simulink library "pneAux_rebuild_generic_std"  (R2016a)
settings: Solver=VariableStepAuto  StartTime=0.0  StopTime=10.0  RelTol=1e-3
undefined symbols (not defined in the file): sMP
(part 1 of 2)
settings Model: Creator=CAB  LastModifiedBy=CAB
settings GRTTargetCC: GeneratePreprocessorConditionals=Use local settings

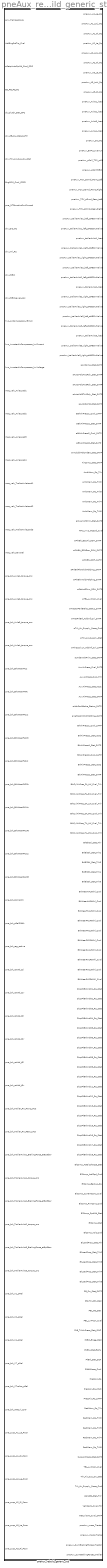
== system pneAux_rebuild_generic_std ==
  pneAux_rebuild_generic_std : Subsystem  mask{s1=sMP.ctrl.pneAux.settings_iMode, s2=sMP.ctrl.pneAux.settings_dt, initCmd='Parameters_pneAux_rebuild_generic_std_sf', p1=sMP.ctrl.pneAux.out.aAirComp_Stat_SATP, p2=sMP.ctrl.pneAux.out.aAutoMd1To2Rdy_Stat_SATP, p3=sMP.ctrl.pneAux.out.aAutoMd1To3Rdy_Stat_SATP, p4=sMP.ctrl.pneAux.out.aAutoMd3To1Rdy_Stat_SATP, p5=sMP.ctrl.pneAux.out.aAutoOpMd_Stat_SATP, p6=sMP.ctrl.pneAux.out.aBrkAirPress1_Cval_SATP, p7=sMP.ctrl.pneAux.out.aBrkAirPress1_Stat_SATP, p8=sMP.ctrl.pneAux.out.aBrkAirPress2_Cval_SATP, p9=sMP.ctrl.pneAux.out.aBrkAirPress2_Stat_SATP, p10=sMP.ctrl.pneAux.in.ActlEngPctTrq_Cval, p11=sMP.ctrl.pneAux.out.aImplsblMdCmdErr_Stat_SATP, p12=sMP.ctrl.pneAux.out.AirComp_Stat_SATP, p13=sMP.ctrl.pneAux.out.AmbWarn_Rq_Trlr2, p14=sMP.ctrl.pneAux.out.AmbWarn_Rq_Trlr3, p15=sMP.ctrl.pneAux.out.AmbWarn_Rq_Trlr4, p16=sMP.ctrl.pneAux.out.AmbWarn_Rq_Trlr5, p17=sMP.ctrl.pneAux.out.AmbWarn_Rq_Trlr, p18=sMP.ctrl.pneAux.out.aOverVoltPrim_Stat_SATP, p19=sMP.ctrl.pneAux.out.API2_Inv2_RqSpd_Cval, p20=sMP.ctrl.pneAux.out.aPrkBrk_ECUAir_SOH_SATP, p21=sMP.ctrl.pneAux.out.aPrkBrk_ECUGen_SOH_SATP, p22=sMP.ctrl.pneAux.out.aPrkBrk_SOH_SATP, p23=sMP.ctrl.pneAux.out.aPrkBrkFltIntrlckMdChng_SATP, p24=sMP.ctrl.pneAux.out.aPrkBrkIntrlckMdChng_SATP, p25=sMP.ctrl.pneAux.in.aSatpAutoOpMd_Cmd_SDS, p26=sMP.ctrl.pneAux.out.aSdsIntfPrim_SOH_SATP, p27=sMP.ctrl.pneAux.out.aTBL_LvrPosn_Cval, p28=sMP.ctrl.pneAux.ATBVehicleParameter, p29=sMP.ctrl.pneAux.out.aTractorParkBrake_Status_SATP, p30=sMP.ctrl.pneAux.out.aTrctrPrkBrk_AddInf_Cvl_SATP, p31=sMP.ctrl.pneAux.out.aTrlr_Air_Supply_Press_Cval, p32=sMP.ctrl.pneAux.out.aTrlr_Air_Supply_Stat, p33=sMP.ctrl.pneAux.out.aTrlrSpplyLn_AddInf_Cvl_SATP, p34=sMP.ctrl.pneAux.out.aUnderVoltPrim_Stat_SATP, p35=sMP.ctrl.pneAux.out.AuxAirPress_Cval_SATP, p36=sMP.ctrl.pneAux.out.AuxAirPress_Cval_Trlr, p37=sMP.ctrl.pneAux.out.AuxAirPress_Stat_ICUC, p38=sMP.ctrl.pneAux.out.AuxAirPress_Stat_SATP, p39=sMP.ctrl.pneAux.out.aVehParkBrake_Status_SATP, p40=sMP.ctrl.pneAux.out.aVehSpdIntrlckMdChng_SATP, p41=sMP.ctrl.pneAux.out.BrkAirPress1_Cval_SATP, p42=sMP.ctrl.pneAux.out.BrkAirPress1_Stat_ICUC, p43=sMP.ctrl.pneAux.out.BrkAirPress1_Stat_SATP, p44=sMP.ctrl.pneAux.out.BrkAirPress2_Cval_SATP, p45=sMP.ctrl.pneAux.out.BrkAirPress2_Stat_ICUC, p46=sMP.ctrl.pneAux.out.BrkAirPress2_Stat_SATP, p47=sMP.ctrl.pneAux.out.BrkCylAirPres_FA_LW_Cval_Trlr, p48=sMP.ctrl.pneAux.out.BrkCylAirPres_FA_RW_Cval_Trlr, p49=sMP.ctrl.pneAux.out.BrkCylAirPres_SA_LW_Cval_Trlr, p50=sMP.ctrl.pneAux.out.BrkCylAirPres_SA_RW_Cval_Trlr, p51=sMP.ctrl.pneAux.out.BrkCylAirPres_TA_LW_Cval_Trlr, p52=sMP.ctrl.pneAux.out.BrkCylAirPres_TA_RW_Cval_Trlr, p53=sMP.ctrl.pneAux.out.BrkElCtrl_Stat_Trlr2, p54=sMP.ctrl.pneAux.out.BrkElCtrl_Stat_Trlr3, p55=sMP.ctrl.pneAux.out.BrkElCtrl_Stat_Trlr4, p56=sMP.ctrl.pneAux.out.BrkElCtrl_Stat_Trlr5, p57=sMP.ctrl.pneAux.out.BrkElCtrl_Stat_Trlr, p58=sMP.ctrl.pneAux.out.BrkWearAALtWhl_Cval, p59=sMP.ctrl.pneAux.out.BrkWearAARtWhl_Cval, p60=sMP.ctrl.pneAux.out.BrkWearFA1LtWhl_Cval, p61=sMP.ctrl.pneAux.out.BrkWearFA1RtWhl_Cval, p62=sMP.ctrl.pneAux.out.BrkWearFA2LtWhl_Cval, p63=sMP.ctrl.pneAux.out.BrkWearFA2RtWhl_Cval, p64=sMP.ctrl.pneAux.out.BrkWearRA1LtWhl_Cval, p65=sMP.ctrl.pneAux.out.BrkWearRA1RtWhl_Cval, p66=sMP.ctrl.pneAux.out.BrkWearRA2LtWhl_Cval, p67=sMP.ctrl.pneAux.out.BrkWearRA2RtWhl_Cval, p68=sMP.ctrl.pneAux.in.BS_PB_Fct_Rq, p69=sMP.ctrl.pneAux.in.ch_Clutch_Stat_CPC, p70=sMP.ctrl.pneAux.out.DispPkBrkInd01_Rq_Stat, p71=sMP.ctrl.pneAux.out.DispPkBrkInd02_Rq_Stat, p72=sMP.ctrl.pneAux.out.DispPkBrkInd03_Rq_Stat, p73=sMP.ctrl.pneAux.out.DispPkBrkInd04_Rq_Stat, p74=sMP.ctrl.pneAux.out.DispPkBrkInd05_Rq_Stat, p75=sMP.ctrl.pneAux.out.DispPkBrkInd06_Rq_Stat, p76=sMP.ctrl.pneAux.out.DispPkBrkInd07_Rq_Stat, p77=sMP.ctrl.pneAux.out.DispPkBrkInd08_Rq_Stat, p78=sMP.ctrl.pneAux.out.DispPkBrkInd09_Rq_Stat, p79=sMP.ctrl.pneAux.out.DispPkBrkInd10_Rq_Stat, p80=sMP.ctrl.pneAux.out.DispPkBrkInd11_Rq_Stat, p81=sMP.ctrl.pneAux.out.DispPkBrkInd12_Rq_Stat, p82=sMP.ctrl.pneAux.out.DispPkBrkInd13_Rq_Stat, p83=sMP.ctrl.pneAux.out.DispPkBrkInd14_Rq_Stat, p84=sMP.ctrl.pneAux.out.DispPkBrkInd15_Rq_Stat, p85=sMP.ctrl.pneAux.out.DispPkBrkInd16_Rq_Stat, p86=sMP.ctrl.pneAux.out.DispPkBrkInd17_Rq_Stat, p87=sMP.ctrl.pneAux.out.DispPkBrkInd18_Rq_Stat, p88=sMP.ctrl.pneAux.in.drv_DrS_Rq, p89=sMP.ctrl.pneAux.in.drv_Knl_Rq, p90=sMP.ctrl.pneAux.in.drv_PB_Sw_Stat_SATP, p91=sMP.ctrl.pneAux.in.drv_PkBrk, p92=sMP.ctrl.pneAux.in.drv_PkBrkLever_pos, p93=sMP.ctrl.pneAux.in.drv_Trlr_Air_Sup_Sw_Stat, p94=sMP.ctrl.pneAux.out.ElComp_ActDischarge_Stat, p95=sMP.ctrl.pneAux.out.ElComp_ActlSpd_Cval, p96=sMP.ctrl.pneAux.out.ElComp_Backup_Rq, p97=sMP.ctrl.pneAux.out.ElComp_CurrentCons_Cval, p98=sMP.ctrl.pneAux.out.ElComp_PwrCons_Cval, p99=sMP.ctrl.pneAux.out.ElComp_SpdMd_Stat, p100=sMP.ctrl.pneAux.out.ElComp_Stat, p101=sMP.ctrl.pneAux.out.ElComp_Volt_Cval, p102=sMP.ctrl.pneAux.out.ElLoadProp_Stat_Trlr2, p103=sMP.ctrl.pneAux.out.ElLoadProp_Stat_Trlr3, p104=sMP.ctrl.pneAux.out.ElLoadProp_Stat_Trlr4, p105=sMP.ctrl.pneAux.out.ElLoadProp_Stat_Trlr5, p106=sMP.ctrl.pneAux.out.ElLoadProp_Stat_Trlr, p107=sMP.ctrl.pneAux.in.EngRPM_Cval_CPC3, p108=sMP.ctrl.pneAux.in.env_Temperature, p109=sMP.ctrl.pneAux.epsLevel, p110=sMP.ctrl.pneAux.veh.flagTrailerABS, p111=sMP.ctrl.pneAux.in.hvs_AirCompressor_nEmot, p112=sMP.ctrl.pneAux.in.hvs_InverterAirCompressor_hvCurrent, p113=sMP.ctrl.pneAux.in.hvs_InverterAirCompressor_hvVoltage, p114=sMP.ctrl.pneAux.kneelingLevel, p115=sMP.ctrl.pneAux.LP_rpmHigh, p116=sMP.ctrl.pneAux.LP_rpmLow, p117=sMP.ctrl.pneAux.in.mec_veh_AxleLoad1, p118=sMP.ctrl.pneAux.in.mec_veh_AxleLoad2, p119=sMP.ctrl.pneAux.in.mec_veh_AxleLoad3, p120=sMP.ctrl.pneAux.in.mec_veh_AxleLoad4, p121=sMP.ctrl.pneAux.in.mec_veh_TrailerAxleLoad1, p122=sMP.ctrl.pneAux.in.mec_veh_TrailerAxleLoad2, p123=sMP.ctrl.pneAux.in.mec_veh_TrailerAxleLoad3, p124=sMP.ctrl.pneAux.in.mec_veh_transVel, p125=sMP.ctrl.pneAux.MTBVehicleParameter, p126=sMP.ctrl.pneAux.out.PB_Sw_Stat_SATP, p127=sMP.ctrl.pneAux.out.PB_Trlr_Ctrl_Stat, p128=sMP.ctrl.pneAux.out.PBL_Fct_Stat, p129=sMP.ctrl.pneAux.out.PBL_LvrPosn_Cval, p130=sMP.ctrl.pneAux.out.PkB_TrlrAirPress_Stat_ICUC, p131=sMP.ctrl.pneAux.out.PkBrk_Engg_Stat, p132=sMP.ctrl.pneAux.out.PkBrk_Stat_EAPU, p133=sMP.ctrl.pneAux.out.PkBrk_Stat_SCH, p134=sMP.ctrl.pneAux.out.PkBrkPress_Cval, p135=sMP.ctrl.pneAux.in.pne_brk_Axle1_torque_sns, p136=sMP.ctrl.pneAux.in.pne_brk_Axle2_torque_sns, p137=sMP.ctrl.pneAux.in.pne_brk_Axle3_torque_sns, p138=sMP.ctrl.pneAux.in.pne_brk_Axle4_torque_sns, p139=sMP.ctrl.pneAux.in.pne_brk_BrkWearAALt, p140=sMP.ctrl.pneAux.in.pne_brk_BrkWearAARt, p141=sMP.ctrl.pneAux.in.pne_brk_BrkWearFA1Lt, p142=sMP.ctrl.pneAux.in.pne_brk_BrkWearFA1Rt, p143=sMP.ctrl.pneAux.in.pne_brk_BrkWearFA2Lt, p144=sMP.ctrl.pneAux.in.pne_brk_BrkWearFA2Rt, p145=sMP.ctrl.pneAux.in.pne_brk_BrkWearRA1Lt, p146=sMP.ctrl.pneAux.in.pne_brk_BrkWearRA1Rt, p147=sMP.ctrl.pneAux.in.pne_brk_BrkWearRA2Lt, p148=sMP.ctrl.pneAux.in.pne_brk_BrkWearRA2Rt, p149=sMP.ctrl.pneAux.in.pne_brk_CompON, p150=sMP.ctrl.pneAux.in.pne_brk_pRelPkBrk, p151=sMP.ctrl.pneAux.in.pne_brk_reg_active, p152=sMP.ctrl.pneAux.in.pne_brk_rotVel_t1l, p153=sMP.ctrl.pneAux.in.pne_brk_rotVel_t1r, p154=sMP.ctrl.pneAux.in.pne_brk_rotVel_t2l, p155=sMP.ctrl.pneAux.in.pne_brk_rotVel_t2r, p156=sMP.ctrl.pneAux.in.pne_brk_rotVel_t3l, p157=sMP.ctrl.pneAux.in.pne_brk_rotVel_t3r, p158=sMP.ctrl.pneAux.in.pne_brk_Trailer_RV_Front_pAct, p159=sMP.ctrl.pneAux.in.pne_brk_Trailer_RV_Rear_pAct, p160=sMP.ctrl.pneAux.in.pne_brk_TrailerAxle1_BrakingForce_at8p5bar, p161=sMP.ctrl.pneAux.in.pne_brk_TrailerAxle1_torque_sns, p162=sMP.ctrl.pneAux.in.pne_brk_TrailerAxle2_BrakingForce_at8p5bar, p163=sMP.ctrl.pneAux.in.pne_brk_TrailerAxle2_torque_sns, p164=sMP.ctrl.pneAux.in.pne_brk_TrailerAxle3_BrakingForce_at8p5bar, p165=sMP.ctrl.pneAux.in.pne_brk_TrailerAxle3_torque_sns, p166=sMP.ctrl.pneAux.in.pne_brk_V1_pRel, p167=sMP.ctrl.pneAux.in.pne_brk_V2_pRel, p168=sMP.ctrl.pneAux.in.pne_brk_V4_pRel, p169=sMP.ctrl.pneAux.in.pne_brk_V7_pRel, p170=sMP.ctrl.pneAux.in.pne_brk_VTrailer_pRel, p171=sMP.ctrl.pneAux.in.pne_brk_WetLvl_Cntr, p172=sMP.ctrl.pneAux.in.pne_MTBmodusSwAllowed, p173=sMP.ctrl.pneAux.in.pne_susp_A1_Le_Posn, p174=sMP.ctrl.pneAux.in.pne_susp_A1_Ri_Posn, p175=sMP.ctrl.pneAux.in.pne_susp_A2_Le_Posn, p176=sMP.ctrl.pneAux.in.pne_susp_A2_Ri_Posn, p177=sMP.ctrl.pneAux.in.pne_susp_A3_Le_Posn, p178=sMP.ctrl.pneAux.in.pne_susp_A3_Ri_Posn, p179=sMP.ctrl.pneAux.out.pneAux_A1_Le_Rq, p180=sMP.ctrl.pneAux.out.pneAux_A1_LoLi_Rq, p181=sMP.ctrl.pneAux.out.pneAux_A1_Ri_Rq, p182=sMP.ctrl.pneAux.out.pneAux_A2_Le_Rq, p183=sMP.ctrl.pneAux.out.pneAux_A2_LoLi_Rq, p184=sMP.ctrl.pneAux.out.pneAux_A2_Ri_Rq, p185=sMP.ctrl.pneAux.out.pneAux_A3_Le_Rq, p186=sMP.ctrl.pneAux.out.pneAux_A3_LoLi_Rq, p187=sMP.ctrl.pneAux.out.pneAux_A3_Ri_Rq, p188=sMP.ctrl.pneAux.out.pneAux_Axle1_load, p189=sMP.ctrl.pneAux.out.pneAux_Axle2_load, p190=sMP.ctrl.pneAux.out.pneAux_Axle3_load, p191=sMP.ctrl.pneAux.out.pneAux_Axle4_load, p192=sMP.ctrl.pneAux.out.pneAux_Drs_Rq, p193=sMP.ctrl.pneAux.out.pneAux_EAPU_overrun, p194=sMP.ctrl.pneAux.out.pneAux_mass_Tractor, p195=sMP.ctrl.pneAux.out.pneAux_mass_Trailer, p196=sMP.ctrl.pneAux.out.pneAux_pSoll_TCV_p43, p197=sMP.ctrl.pneAux.out.pneAux_pSollPkBrk, p198=sMP.ctrl.pneAux.out.pneAux_SumBrakingForces_Tractor, p199=sMP.ctrl.pneAux.out.pneAux_SumBrakingForces_Trailer, p200=sMP.ctrl.pneAux.out.pneAux_TCV_pDmd_Front_Left, p201=sMP.ctrl.pneAux.out.pneAux_TCV_pDmd_Front_Right, p202=sMP.ctrl.pneAux.out.pneAux_TCV_pDmd_Rear_Left, p203=sMP.ctrl.pneAux.out.pneAux_TCV_pDmd_Rear_Right, p204=sMP.ctrl.pneAux.out.pneAux_trailerAxle1_left_stABSInValve, p205=sMP.ctrl.pneAux.out.pneAux_trailerAxle1_left_stABSOutValve, p206=sMP.ctrl.pneAux.out.pneAux_trailerAxle1_load, p207=sMP.ctrl.pneAux.out.pneAux_trailerAxle1_right_stABSInValve, p208=sMP.ctrl.pneAux.out.pneAux_trailerAxle1_right_stABSOutValve, p209=sMP.ctrl.pneAux.out.pneAux_trailerAxle2_left_stABSInValve, p210=sMP.ctrl.pneAux.out.pneAux_trailerAxle2_left_stABSOutValve, p211=sMP.ctrl.pneAux.out.pneAux_trailerAxle2_load, p212=sMP.ctrl.pneAux.out.pneAux_trailerAxle2_right_stABSInValve, p213=sMP.ctrl.pneAux.out.pneAux_trailerAxle2_right_stABSOutValve, p214=sMP.ctrl.pneAux.out.pneAux_trailerAxle3_left_stABSInValve, p215=sMP.ctrl.pneAux.out.pneAux_trailerAxle3_left_stABSOutValve, p216=sMP.ctrl.pneAux.out.pneAux_trailerAxle3_load, p217=sMP.ctrl.pneAux.out.pneAux_trailerAxle3_right_stABSInValve, p218=sMP.ctrl.pneAux.out.pneAux_trailerAxle3_right_stABSOutValve, p219=sMP.ctrl.pneAux.out.PressAir_Rq, p220=sMP.ctrl.pneAux.out.PressAir_Rq_ICUC, p221=sMP.ctrl.pneAux.out.PressAir_Rq_SATP, p222=sMP.ctrl.pneAux.pSwitch_bar, p223=sMP.ctrl.pneAux.veh.rdynFA, p224=sMP.ctrl.pneAux.veh.rdynRA, p225=sMP.ctrl.pneAux.veh.rdynTA, p226=sMP.ctrl.pneAux.out.RedWarn_Rq_Trlr2, p227=sMP.ctrl.pneAux.out.RedWarn_Rq_Trlr3, p228=sMP.ctrl.pneAux.out.RedWarn_Rq_Trlr4, p229=sMP.ctrl.pneAux.out.RedWarn_Rq_Trlr5, p230=sMP.ctrl.pneAux.out.RedWarn_Rq_Trlr, p231=sMP.ctrl.pneAux.veh.stepSize, p232=sMP.ctrl.pneAux.out.SuspAirPress_Stat_SATP, p233=sMP.ctrl.pneAux.out.TBL_LvrPosn_Cval, p234=sMP.ctrl.pneAux.tDelay, p235=sMP.ctrl.pneAux.veh.TrailerABS_L1o, p236=sMP.ctrl.pneAux.veh.TrailerABS_L1v, p237=sMP.ctrl.pneAux.veh.TrailerABS_L2o, p238=sMP.ctrl.pneAux.veh.TrailerABS_L2v, p239=sMP.ctrl.pneAux.veh.TrailerABS_MinusB, p240=sMP.ctrl.pneAux.veh.TrailerABS_PlusB, p241=sMP.ctrl.pneAux.veh.TrailerABS_PlusOB, p242=sMP.ctrl.pneAux.veh.TrailerABS_THe, p243=sMP.ctrl.pneAux.veh.TrailerABS_TPulHold, p244=sMP.ctrl.pneAux.veh.TrailerABS_TPulOpen, p245=sMP.ctrl.pneAux.veh.TrailerABS_vMin_kmh, p246=sMP.ctrl.pneAux.out.Trlr_Air_Sup_Sw_Stat, p247=sMP.ctrl.pneAux.out.Trlr_Air_Supply_Press_Cval, p248=sMP.ctrl.pneAux.out.VehABS_Stat_Trlr, p249=sMP.ctrl.pneAux.out.VehSpd1_Cval_Trlr, p250=sMP.ctrl.pneAux.out.WetLvlCntr_Cval_SATP, p251=sMP.ctrl.pneAux.veh.axleLoadTrailer_kg, p252=sMP.ctrl.pneAux.veh.axleLoadVehicle_kg, p253=sMP.ctrl.pneAux.veh.brkCircuit, p254=sMP.ctrl.pneAux.veh.brkCircuitTrailer, p255=sMP.ctrl.pneAux.veh.flagTrailerControlActive, p256=sMP.ctrl.pneAux.veh.pAppCyl_Trailer, p257=sMP.ctrl.pneAux.veh.speedSensorPosnTrailer}
      mask prompts: s1 "Solver Type: settings_iMode [-]"; s2 "Solver Step Size: settings_dt [s]"; initCmd "Initialization command"; p1 "aAirComp_Stat_SATP, Compressor status: 0,1,2,3 / inactiv, active, err, SNA export=true name=aAirComp_Stat_SATP prio=1 dataSetName=std dataClassType=initIO dataClassName=initIO unit='-' description='Compressor status: 0,1,2,3 / inactiv, active, err, SNA': pneAux.aAirComp_Stat_SATP_0 [-]"; p2 "aAutoMd1To2Rdy_Stat_SATP, L4 - Driver mode: 0,1,2,3 / not ready, ready, reserved, SNA ((ATG) Readiness status of SATP to transition from mode 1 to mode 2) export=true name=aAutoMd1To2Rdy_Stat_SATP prio=1 dataSetName=std dataClassType=initIO dataClassName=initIO unit='-' description='L4 - Driver mode: 0,1,2,3 / not ready, ready, reserved, SNA ((ATG) Readiness status of SATP to transition from mode 1 to mode 2)': pneAux.aAutoMd1To2Rdy_Stat_SATP_0 [-]"; p3 "aAutoMd1To3Rdy_Stat_SATP, L4 - Driver mode: 0,1,2,3 / not ready, ready, reserved, SNA ((ATG) Readiness status of SATP to transition from mode 1 to mode 3) export=true name=aAutoMd1To3Rdy_Stat_SATP prio=1 dataSetName=std dataClassType=initIO dataClassName=initIO unit='-' description='L4 - Driver mode: 0,1,2,3 / not ready, ready, reserved, SNA ((ATG) Readiness status of SATP to transition from mode 1 to mode 3)': pneAux.aAutoMd1To3Rdy_Stat_SATP_0 [-]"; p4 "aAutoMd3To1Rdy_Stat_SATP, L4 - Driver mode: 0,1,2,3 / not ready, ready, reserved, SNA ((ATG) Readiness status of SATP to transition from mode 3 to mode 1) export=true name=aAutoMd3To1Rdy_Stat_SATP prio=1 dataSetName=std dataClassType=initIO dataClassName=initIO unit='-' description='L4 - Driver mode: 0,1,2,3 / not ready, ready, reserved, SNA ((ATG) Readiness status of SATP to transition from mode 3 to mode 1)': pneAux.aAutoMd3To1Rdy_Stat_SATP_0 [-]"; p5 "aAutoOpMd_Stat_SATP, 0,1,2,3 /  MODE_1 Manual Mode, L4_IFTD SAE L4 with IFTD, L4_NDC SAE L4 with no driver controls, SNA Signal not Available export=true name=aAutoOpMd_Stat_SATP prio=1 dataSetName=std dataClassType=initIO dataClassName=initIO unit='-' description='0,1,2,3 /  MODE_1 Manual Mode, L4_IFTD SAE L4 with IFTD, L4_NDC SAE L4 with no driver controls, SNA Signal not Available': pneAux.aAutoOpMd_Stat_SATP_0 [-]"; p6 "aBrkAirPress1_Cval_SATP (init) export=true name=aBrkAirPress1_Cval_SATP prio=1 dataSetName=std dataClassType=initIO dataClassName=initIO unit=kPa description='aBrkAirPress1_Cval_SATP': pneAux.aBrkAirPress1_Cval_SATP_0 [-]"; p7 "aBrkAirPress1_Stat_SATP (init) export=true name=aBrkAirPress1_Stat_SATP prio=1 dataSetName=std dataClassType=initIO dataClassName=initIO unit=kPa description='aBrkAirPress1_Stat_SATP': pneAux.aBrkAirPress1_Stat_SATP_0 [-]"; p8 "aBrkAirPress2_Cval_SATP (init) export=true name=aBrkAirPress2_Cval_SATP prio=1 dataSetName=std dataClassType=initIO dataClassName=initIO unit=kPa description='aBrkAirPress2_Cval_SATP': pneAux.aBrkAirPress2_Cval_SATP_0 [-]"; p9 "aBrkAirPress2_Stat_SATP (init) export=true name=aBrkAirPress2_Stat_SATP prio=1 dataSetName=std dataClassType=initIO dataClassName=initIO unit=kPa description='aBrkAirPress2_Stat_SATP': pneAux.aBrkAirPress2_Stat_SATP_0 [-]"; p10 "ActlEngPctTrq_Cval (init) export=true name=ActlEngPctTrq_Cval prio=1 dataSetName=std dataClassType=initIO dataClassName=initIO unit='-' description='ActlEngPctTrq_Cval': pneAux.ActlEngPctTrq_Cval_0 [-]"; p11 "aImplsblMdCmdErr_Stat_SATP, 0,1,2,3 /  OK, invalid, reserved, SNA export=true name=aImplsblMdCmdErr_Stat_SATP prio=1 dataSetName=std dataClassType=initIO dataClassName=initIO unit='-' description='0,1,2,3 /  OK, invalid, reserved, SNA': pneAux.aImplsblMdCmdErr_Stat_SATP_0 [-]"; p12 "AirComp_Stat_SATP, Compressor status: 0,1,2,3 / inactiv, active, err, SNA export=true name=AirComp_Stat_SATP prio=1 dataSetName=std dataClassType=initIO dataClassName=initIO unit='-' description='Compressor status: 0,1,2,3 / inactiv, active, err, SNA': pneAux.AirComp_Stat_SATP_0 [-]"; p13 "AmbWarn_Rq_Trlr2,   export=true name=AmbWarn_Rq_Trlr2 prio=1 dataSetName=std dataClassType=initIO dataClassName=initIO unit='-' description=' ': pneAux.AmbWarn_Rq_Trlr2_0 [-]"; p14 "AmbWarn_Rq_Trlr3,   export=true name=AmbWarn_Rq_Trlr3 prio=1 dataSetName=std dataClassType=initIO dataClassName=initIO unit='-' description=' ': pneAux.AmbWarn_Rq_Trlr3_0 [-]"; p15 "AmbWarn_Rq_Trlr4,   export=true name=AmbWarn_Rq_Trlr4 prio=1 dataSetName=std dataClassType=initIO dataClassName=initIO unit='-' description=' ': pneAux.AmbWarn_Rq_Trlr4_0 [-]"; p16 "AmbWarn_Rq_Trlr5,   export=true name=AmbWarn_Rq_Trlr5 prio=1 dataSetName=std dataClassType=initIO dataClassName=initIO unit='-' description=' ': pneAux.AmbWarn_Rq_Trlr5_0 [-]"; p17 "AmbWarn_Rq_Trlr export=true name=AmbWarn_Rq_Trlr prio=1 dataSetName=std dataClassType=initIO dataClassName=initIO unit='-' description='AmbWarn_Rq_Trlr': pneAux.AmbWarn_Rq_Trlr_0 [-]"; p18 "aOverVoltPrim_Stat_SATP, 0,1,2,3 /  OK, overvoltage, reserved, SNA export=true name=aOverVoltPrim_Stat_SATP prio=1 dataSetName=std dataClassType=initIO dataClassName=initIO unit='-' description='0,1,2,3 /  OK, overvoltage, reserved, SNA': pneAux.aOverVoltPrim_Stat_SATP_0 [-]"; p19 "Inverter 2 Requested Speed API2 for air compressor (init) export=true name=API2_Inv2_RqSpd_Cval prio=1 dataSetName=std dataClassType=initIO dataClassName=initIO unit='-' description='Inverter 2 Requested Speed API2 for air compressor (init)': pneAux.API2_Inv2_RqSpd_Cval_0 [-]"; p20 "aPrkBrk_ECUAir_SOH_SATP,  (ATG) ECU  Air management health status: 0 Fully Operational / 1 Partly Operational / 2 Not Operational / 3 SNA export=true name=aPrkBrk_ECUAir_SOH_SATP prio=1 dataSetName=std dataClassType=initIO dataClassName=initIO unit='-' description=' (ATG) ECU  Air management health status: 0 Fully Operational / 1 Partly Operational / 2 Not Operational / 3 SNA': pneAux.aPrkBrk_ECUAir_SOH_SATP_0 [-]"; p21 "aPrkBrk_ECUGen_SOH_SATP,  (ATG) ECU general health status: 0 Fully Operational / 1 Partly Operational / 2 Not Operational / 3 SNA export=true name=aPrkBrk_ECUGen_SOH_SATP prio=1 dataSetName=std dataClassType=initIO dataClassName=initIO unit='-' description=' (ATG) ECU general health status: 0 Fully Operational / 1 Partly Operational / 2 Not Operational / 3 SNA': pneAux.aPrkBrk_ECUGen_SOH_SATP_0 [-]"; p22 "aPrkBrk_SOH_SATP,  (ATG) Parking Brake System Health Status: 0 Fully Operational / 1 Partly Operational / 2 Not Operational / 3 SNA export=true name=aPrkBrk_SOH_SATP prio=1 dataSetName=std dataClassType=initIO dataClassName=initIO unit='-' description=' (ATG) Parking Brake System Health Status: 0 Fully Operational / 1 Partly Operational / 2 Not Operational / 3 SNA': pneAux.aPrkBrk_SOH_SATP_0 [-]"; p23 "aPrkBrkFltIntrlckMdChng_SATP, 0,1,2,3 /  NoT met, met, reserved, SNA ((ATG) Current status in SATP for the Fault interlock for mode change) export=true name=aPrkBrkFltIntrlckMdChng_SATP prio=1 dataSetName=std dataClassType=initIO dataClassName=initIO unit='-' description='0,1,2,3 /  NoT met, met, reserved, SNA ((ATG) Current status in SATP for the Fault interlock for mode change)': pneAux.aPrkBrkFltIntrlckMdChng_SATP_0 [-]"; p24 "aPrkBrkIntrlckMdChng_SATP, 0,1,2,3 /  NoT met, met, reserved, SNA ((ATG) Current status in SATP for the park brake interlock for mode change) export=true name=aPrkBrkIntrlckMdChng_SATP prio=1 dataSetName=std dataClassType=initIO dataClassName=initIO unit='-' description='0,1,2,3 /  NoT met, met, reserved, SNA ((ATG) Current status in SATP for the park brake interlock for mode change)': pneAux.aPrkBrkIntrlckMdChng_SATP_0 [-]"; p25 "aSatpAutoOpMd_Cmd_SDS (init) export=true name=aSatpAutoOpMd_Cmd_SDS prio=1 dataSetName=std dataClassType=initIO dataClassName=initIO unit='-' description='SATP operational mode command by SDS': pneAux.aSatpAutoOpMd_Cmd_SDS_0 [-]"; p26 "aSdsIntfPrim_SOH_SATP,   export=true name=aSdsIntfPrim_SOH_SATP prio=1 dataSetName=std dataClassType=initIO dataClassName=initIO unit='-' description=' ': pneAux.aSdsIntfPrim_SOH_SATP_0 [-]"; p27 "aTBL_LvrPosn_Cval, Lever: 0..100, 101..253,254,255 / 0..100, RES,ERR,SNA export=true name=aTBL_LvrPosn_Cval prio=1 dataSetName=std dataClassType=initIO dataClassName=initIO unit='%' description='Lever: 0..100, 101..253,254,255 / 0..100, RES,ERR,SNA': pneAux.aTBL_LvrPosn_Cval_0 [-]"; p28 "ATBVehicleParameter (0-disabled, 1-enabled) export=true name=ATBVehicleParameter prio=1 dataSetName=pneAux_dummy dataClassType=main dataClassName=main unit='-' description='ATBVehicleParameter (0-disabled, 1-enabled)': pneAux.ATBVehicleParameter [-]"; p29 "aTractorParkBrake_Status_SATP, 0,1,2,6,7 / ENGG Engaged, INT Intermediate Position, DISENGG Disengaged, ERR, SNA ((ATG)  export=true name=aTractorParkBrake_Status_SATP prio=1 dataSetName=std dataClassType=initIO dataClassName=initIO unit='-' description='0,1,2,6,7 / ENGG Engaged, INT Intermediate Position, DISENGG Disengaged, ERR, SNA ((ATG) ': pneAux.aTractorParkBrake_Status_SATP_0 [-]"; p30 "aTrctrPrkBrk_AddInf_Cvl_SATP, 0,1,2,6,7 / DEFLATED Deflated (parked), INT Intermediate, INFLATED Inflated (unparked), ERR, SNA ((ATG)  export=true name=aTrctrPrkBrk_AddInf_Cvl_SATP prio=1 dataSetName=std dataClassType=initIO dataClassName=initIO unit='-' description='0,1,2,6,7 / DEFLATED Deflated (parked), INT Intermediate, INFLATED Inflated (unparked), ERR, SNA ((ATG) ': pneAux.aTrctrPrkBrk_AddInf_Cvl_SATP_0 [-]"; p31 "aTrlr_Air_Supply_Press_Cval, 0..250,251..253,254,255 / 0..2000, RES,ERR,SNA export=true name=aTrlr_Air_Supply_Press_Cval prio=1 dataSetName=std dataClassType=initIO dataClassName=initIO unit='kPa' description='0..250,251..253,254,255 / 0..2000, RES,ERR,SNA': pneAux.aTrlr_Air_Supply_Press_Cval_0 [-]"; p32 "aTrlr_Air_Supply_Stat (init), 0,1,2,3 / SPL supplied, NSPL not supplied, ERR, SAN ((ATG) Trailer Air Supply Current state) export=true name=aTrlr_Air_Supply_Stat prio=1 dataSetName=std dataClassType=initIO dataClassName=initIO unit='-' description='0,1,2,3 / SPL supplied, NSPL not supplied, ERR, SAN ((ATG) Trailer Air Supply Current state)': pneAux.aTrlr_Air_Supply_Stat_0 [-]"; p33 "aTrlrSpplyLn_AddInf_Cvl_SATP, 0,1,2,3 / HIGH_INT Signal integrity High, 1 LOW_INT Signal Integrity low, 2 NO_SENSING no sensing possible, SNA ((ATG) Trailer Supply Line Additional  export=true name=aTrlrSpplyLn_AddInf_Cvl_SATP prio=1 dataSetName=std dataClassType=initIO dataClassName=initIO unit='-' description='0,1,2,3 / HIGH_INT Signal integrity High, 1 LOW_INT Signal Integrity low, 2 NO_SENSING no sensing possible, SNA ((ATG) Trailer Supply Line Additional ': pneAux.aTrlrSpplyLn_AddInf_Cvl_SATP_0 [-]"; p34 "aUnderVoltPrim_Stat_SATP, (ATG) Primary Under Voltage Status SBSP export=true name=aUnderVoltPrim_Stat_SATP prio=1 dataSetName=std dataClassType=initIO dataClassName=initIO unit='-' description='(ATG) Primary Under Voltage Status SBSP': pneAux.aUnderVoltPrim_Stat_SATP_0 [-]"; p35 "AuxAirPress_Cval_SATP (init) export=true name=AuxAirPress_Cval_SATP prio=1 dataSetName=std dataClassType=initIO dataClassName=initIO unit=kPa description='AuxAirPress_Cval_SATP': pneAux.AuxAirPress_Cval_SATP_0 [-]"; p36 "AuxAirPress_Cval_Trlr (init) export=true name=AuxAirPress_Cval_Trlr prio=1 dataSetName=std dataClassType=initIO dataClassName=initIO unit=kPa description='AuxAirPress_Cval_Trlr': pneAux.AuxAirPress_Cval_Trlr_0 [-]"; p37 "AuxAirPress_Stat_ICUC (init) export=true name=AuxAirPress_Stat_ICUC prio=1 dataSetName=std dataClassType=initIO dataClassName=initIO unit=kPa description='AuxAirPress_Stat_ICUC': pneAux.AuxAirPress_Stat_ICUC_0 [-]"; p38 "AuxAirPress_Stat_SATP (init) export=true name=AuxAirPress_Stat_SATP prio=1 dataSetName=std dataClassType=initIO dataClassName=initIO unit=kPa description='AuxAirPress_Stat_SATP': pneAux.AuxAirPress_Stat_SATP_0 [-]"; p39 "aVehParkBrake_Status_SATP, Parking Brake Status entire vehicle: 0,1,2,3,6,7 / SAFE_PARK Safety Parked, NO_DRIVEOFF Drive-Off Inhibited, SAFE_DRIVEOFF_CBN Safe Drive-Off Combined, SAFE_DRIVEOFF_BT Safe Drive-Off- Bobtail, ERR, SNA ((ATG)  export=true name=aVehParkBrake_Status_SATP prio=1 dataSetName=std dataClassType=initIO dataClassName=initIO unit='-' description='Parking Brake Status entire vehicle: 0,1,2,3,6,7 / SAFE_PARK Safety Parked, NO_DRIVEOFF Drive-Off Inhibited, SAFE_DRIVEOFF_CBN Safe Drive-Off Combined, SAFE_DRIVEOFF_BT Safe Drive-Off- Bobtail, ERR, SNA ((ATG) ': pneAux.aVehParkBrake_Status_SATP_0 [-]"; p40 "aVehSpdIntrlckMdChng_SATP, 0,1,2,3 / NoT met, met, reserved, SNA ((ATG) Current status in SATP for the vehicle speed interlock for mode change export=true name=aVehSpdIntrlckMdChng_SATP prio=1 dataSetName=std dataClassType=initIO dataClassName=initIO unit='-' description='0,1,2,3 / NoT met, met, reserved, SNA ((ATG) Current status in SATP for the vehicle speed interlock for mode change': pneAux.aVehSpdIntrlckMdChng_SATP_0 [-]"; p41 "BrkAirPress1_Cval_SATP (init) export=true name=BrkAirPress1_Cval_SATP prio=1 dataSetName=std dataClassType=initIO dataClassName=initIO unit=kPa description='BrkAirPress1_Cval_SATP': pneAux.BrkAirPress1_Cval_SATP_0 [-]"; p42 "BrkAirPress1_Stat_ICUC (init) export=true name=BrkAirPress1_Stat_ICUC prio=1 dataSetName=std dataClassType=initIO dataClassName=initIO unit=kPa description='BrkAirPress1_Stat_ICUC': pneAux.BrkAirPress1_Stat_ICUC_0 [-]"; p43 "BrkAirPress1_Stat_SATP (init) export=true name=BrkAirPress1_Stat_SATP prio=1 dataSetName=std dataClassType=initIO dataClassName=initIO unit=kPa description='BrkAirPress1_Stat_SATP': pneAux.BrkAirPress1_Stat_SATP_0 [-]"; p44 "BrkAirPress2_Cval_SATP (init) export=true name=BrkAirPress2_Cval_SATP prio=1 dataSetName=std dataClassType=initIO dataClassName=initIO unit=kPa description='BrkAirPress2_Cval_SATP': pneAux.BrkAirPress2_Cval_SATP_0 [-]"; p45 "BrkAirPress2_Stat_ICUC (init) export=true name=BrkAirPress2_Stat_ICUC prio=1 dataSetName=std dataClassType=initIO dataClassName=initIO unit=kPa description='BrkAirPress2_Stat_ICUC': pneAux.BrkAirPress2_Stat_ICUC_0 [-]"; p46 "BrkAirPress2_Stat_SATP (init) export=true name=BrkAirPress2_Stat_SATP prio=1 dataSetName=std dataClassType=initIO dataClassName=initIO unit=kPa description='BrkAirPress2_Stat_SATP': pneAux.BrkAirPress2_Stat_SATP_0 [-]"; p47 "Trailer brake pressur first axle left wheel (init) export=true name=BrkCylAirPres_FA_LW_Cval_Trlr prio=1 dataSetName=std dataClassType=initIO dataClassName=initIO unit=kPa description='Trailer brake pressur first axle left wheel': pneAux.BrkCylAirPres_FA_LW_Cval_Trlr_0 [-]"; p48 "Trailer brake pressur first axle right wheel (init) export=true name=BrkCylAirPres_FA_RW_Cval_Trlr prio=1 dataSetName=std dataClassType=initIO dataClassName=initIO unit=kPa description='Trailer brake pressur first axle right wheel': pneAux.BrkCylAirPres_FA_RW_Cval_Trlr_0 [-]"; p49 "Trailer brake pressur second axle left wheel (init) export=true name=BrkCylAirPres_SA_LW_Cval_Trlr prio=1 dataSetName=std dataClassType=initIO dataClassName=initIO unit=kPa description='Trailer brake pressur second axle left wheel': pneAux.BrkCylAirPres_SA_LW_Cval_Trlr_0 [-]"; p50 "Trailer brake pressur second axle right wheel (init) export=true name=BrkCylAirPres_SA_RW_Cval_Trlr prio=1 dataSetName=std dataClassType=initIO dataClassName=initIO unit=kPa description='Trailer brake pressur second axle right wheel': pneAux.BrkCylAirPres_SA_RW_Cval_Trlr_0 [-]"; p51 "Trailer brake pressur third axle left wheel (init) export=true name=BrkCylAirPres_TA_LW_Cval_Trlr prio=1 dataSetName=std dataClassType=initIO dataClassName=initIO unit=kPa description='Trailer brake pressur third axle left wheel': pneAux.BrkCylAirPres_TA_LW_Cval_Trlr_0 [-]"; p52 "Trailer brake pressur third axle right wheel (init) export=true name=BrkCylAirPres_TA_RW_Cval_Trlr prio=1 dataSetName=std dataClassType=initIO dataClassName=initIO unit=kPa description='Trailer brake pressur third axle right wheel': pneAux.BrkCylAirPres_TA_RW_Cval_Trlr_0 [-]"; p53 "BrkElCtrl_Stat_Trlr2,   export=true name=BrkElCtrl_Stat_Trlr2 prio=1 dataSetName=std dataClassType=initIO dataClassName=initIO unit='-' description=' ': pneAux.BrkElCtrl_Stat_Trlr2_0 [-]"; p54 "BrkElCtrl_Stat_Trlr3,   export=true name=BrkElCtrl_Stat_Trlr3 prio=1 dataSetName=std dataClassType=initIO dataClassName=initIO unit='-' description=' ': pneAux.BrkElCtrl_Stat_Trlr3_0 [-]"; p55 "BrkElCtrl_Stat_Trlr4,   export=true name=BrkElCtrl_Stat_Trlr4 prio=1 dataSetName=std dataClassType=initIO dataClassName=initIO unit='-' description=' ': pneAux.BrkElCtrl_Stat_Trlr4_0 [-]"; p56 "BrkElCtrl_Stat_Trlr5,   export=true name=BrkElCtrl_Stat_Trlr5 prio=1 dataSetName=std dataClassType=initIO dataClassName=initIO unit='-' description=' ': pneAux.BrkElCtrl_Stat_Trlr5_0 [-]"; p57 "BrkElCtrl_Stat_Trlr export=true name=BrkElCtrl_Stat_Trlr prio=1 dataSetName=std dataClassType=initIO dataClassName=initIO unit='-' description='BrkElCtrl_Stat_Trlr': pneAux.BrkElCtrl_Stat_Trlr_0 [-]"; p58 "BrkWearAALtWhl_Cval export=true name=BrkWearAALtWhl_Cval prio=1 dataSetName=std dataClassType=initIO dataClassName=initIO unit='%' description='BrkWearAALtWhl_Cval': pneAux.BrkWearAALtWhl_Cval_0 [-]"; p59 "BrkWearAARtWhl_Cval export=true name=BrkWearAARtWhl_Cval prio=1 dataSetName=std dataClassType=initIO dataClassName=initIO unit='%' description='BrkWearAARtWhl_Cval': pneAux.BrkWearAARtWhl_Cval_0 [-]"; p60 "BrkWearFA1LtWhl_Cval export=true name=BrkWearFA1LtWhl_Cval prio=1 dataSetName=std dataClassType=initIO dataClassName=initIO unit='%' description='BrkWearFA1LtWhl_Cval': pneAux.BrkWearFA1LtWhl_Cval_0 [-]"; p61 "BrkWearFA1LtWhl_Cval export=true name=BrkWearFA1RtWhl_Cval prio=1 dataSetName=std dataClassType=initIO dataClassName=initIO unit='%' description='BrkWearFA1RtWhl_Cval': pneAux.BrkWearFA1RtWhl_Cval_0 [-]"; p62 "BrkWearFA1LtWhl_Cval export=true name=BrkWearFA2LtWhl_Cval prio=1 dataSetName=std dataClassType=initIO dataClassName=initIO unit='%' description='BrkWearFA2LtWhl_Cval': pneAux.BrkWearFA2LtWhl_Cval_0 [-]"; p63 "BrkWearFA1LtWhl_Cval export=true name=BrkWearFA2RtWhl_Cval prio=1 dataSetName=std dataClassType=initIO dataClassName=initIO unit='%' description='BrkWearFA2RtWhl_Cval': pneAux.BrkWearFA2RtWhl_Cval_0 [-]"; p64 "BrkWearRA1LtWhl_Cval export=true name=BrkWearRA1LtWhl_Cval prio=1 dataSetName=std dataClassType=initIO dataClassName=initIO unit='%' description='BrkWearRA1LtWhl_Cval': pneAux.BrkWearRA1LtWhl_Cval_0 [-]"; p65 "BrkWearRA1LtWhl_Cval export=true name=BrkWearRA1RtWhl_Cval prio=1 dataSetName=std dataClassType=initIO dataClassName=initIO unit='%' description='BrkWearRA1RtWhl_Cval': pneAux.BrkWearRA1RtWhl_Cval_0 [-]"; p66 "BrkWearRA1LtWhl_Cval export=true name=BrkWearRA2LtWhl_Cval prio=1 dataSetName=std dataClassType=initIO dataClassName=initIO unit='%' description='BrkWearRA2LtWhl_Cval': pneAux.BrkWearRA2LtWhl_Cval_0 [-]"; p67 "BrkWearRA1LtWhl_Cval export=true name=BrkWearRA2RtWhl_Cval prio=1 dataSetName=std dataClassType=initIO dataClassName=initIO unit='%' description='BrkWearRA2RtWhl_Cval': pneAux.BrkWearRA2RtWhl_Cval_0 [-]"; p68 "BS_PB_Fct_Rq (init) export=true name=BS_PB_Fct_Rq prio=1 dataSetName=std dataClassType=initIO dataClassName=initIO unit='-' description='BS_PB_Fct_Rq': pneAux.BS_PB_Fct_Rq_0 [-]"; p69 "ch_Clutch_Stat_CPC (init) export=true name=ch_Clutch_Stat_CPC prio=1 dataSetName=std dataClassType=initIO dataClassName=initIO unit='-' description='ch_Clutch_Stat_CPC (init)': pneAux.ch_Clutch_Stat_CPC_0 [-]"; p70 "DispPkBrkInd01_Rq_Stat, 0,1,2,3 / not requested, requested, res, sna (Display Park(ing) Brake(ing) Indication/Indicator 01 Requested state Current state export=true name=DispPkBrkInd01_Rq_Stat prio=1 dataSetName=std dataClassType=initIO dataClassName=initIO unit='-' description='0,1,2,3 / not requested, requested, res, sna (Display Park(ing) Brake(ing) Indication/Indicator 01 Requested state Current state': pneAux.DispPkBrkInd01_Rq_Stat_0 [-]"; p71 "DispPkBrkInd02_Rq_Stat, 0,1,2,3 / not requested, requested, res, sna (Display Park(ing) Brake(ing) Indication/Indicator 01 Requested state Current state export=true name=DispPkBrkInd02_Rq_Stat prio=1 dataSetName=std dataClassType=initIO dataClassName=initIO unit='-' description='0,1,2,3 / not requested, requested, res, sna (Display Park(ing) Brake(ing) Indication/Indicator 01 Requested state Current state': pneAux.DispPkBrkInd02_Rq_Stat_0 [-]"; p72 "DispPkBrkInd03_Rq_Stat, 0,1,2,3 / not requested, requested, res, sna (Display Park(ing) Brake(ing) Indication/Indicator 01 Requested state Current state export=true name=DispPkBrkInd03_Rq_Stat prio=1 dataSetName=std dataClassType=initIO dataClassName=initIO unit='-' description='0,1,2,3 / not requested, requested, res, sna (Display Park(ing) Brake(ing) Indication/Indicator 01 Requested state Current state': pneAux.DispPkBrkInd03_Rq_Stat_0 [-]"; p73 "DispPkBrkInd04_Rq_Stat, 0,1,2,3 / not requested, requested, res, sna (Display Park(ing) Brake(ing) Indication/Indicator 01 Requested state Current state export=true name=DispPkBrkInd04_Rq_Stat prio=1 dataSetName=std dataClassType=initIO dataClassName=initIO unit='-' description='0,1,2,3 / not requested, requested, res, sna (Display Park(ing) Brake(ing) Indication/Indicator 01 Requested state Current state': pneAux.DispPkBrkInd04_Rq_Stat_0 [-]"; p74 "DispPkBrkInd05_Rq_Stat, 0,1,2,3 / not requested, requested, res, sna (Display Park(ing) Brake(ing) Indication/Indicator 01 Requested state Current state export=true name=DispPkBrkInd05_Rq_Stat prio=1 dataSetName=std dataClassType=initIO dataClassName=initIO unit='-' description='0,1,2,3 / not requested, requested, res, sna (Display Park(ing) Brake(ing) Indication/Indicator 01 Requested state Current state': pneAux.DispPkBrkInd05_Rq_Stat_0 [-]"; p75 "DispPkBrkInd06_Rq_Stat, 0,1,2,3 / not requested, requested, res, sna (Display Park(ing) Brake(ing) Indication/Indicator 01 Requested state Current state export=true name=DispPkBrkInd06_Rq_Stat prio=1 dataSetName=std dataClassType=initIO dataClassName=initIO unit='-' description='0,1,2,3 / not requested, requested, res, sna (Display Park(ing) Brake(ing) Indication/Indicator 01 Requested state Current state': pneAux.DispPkBrkInd06_Rq_Stat_0 [-]"; p76 "DispPkBrkInd07_Rq_Stat, 0,1,2,3 / not requested, requested, res, sna (Display Park(ing) Brake(ing) Indication/Indicator 01 Requested state Current state export=true name=DispPkBrkInd07_Rq_Stat prio=1 dataSetName=std dataClassType=initIO dataClassName=initIO unit='-' description='0,1,2,3 / not requested, requested, res, sna (Display Park(ing) Brake(ing) Indication/Indicator 01 Requested state Current state': pneAux.DispPkBrkInd07_Rq_Stat_0 [-]"; p77 "DispPkBrkInd08_Rq_Stat, 0,1,2,3 / not requested, requested, res, sna (Display Park(ing) Brake(ing) Indication/Indicator 01 Requested state Current state export=true name=DispPkBrkInd08_Rq_Stat prio=1 dataSetName=std dataClassType=initIO dataClassName=initIO unit='-' description='0,1,2,3 / not requested, requested, res, sna (Display Park(ing) Brake(ing) Indication/Indicator 01 Requested state Current state': pneAux.DispPkBrkInd08_Rq_Stat_0 [-]"; p78 "DispPkBrkInd09_Rq_Stat, 0,1,2,3 / not requested, requested, res, sna (Display Park(ing) Brake(ing) Indication/Indicator 01 Requested state Current state export=true name=DispPkBrkInd09_Rq_Stat prio=1 dataSetName=std dataClassType=initIO dataClassName=initIO unit='-' description='0,1,2,3 / not requested, requested, res, sna (Display Park(ing) Brake(ing) Indication/Indicator 01 Requested state Current state': pneAux.DispPkBrkInd09_Rq_Stat_0 [-]"; p79 "DispPkBrkInd10_Rq_Stat, 0,1,2,3 / not requested, requested, res, sna (Display Park(ing) Brake(ing) Indication/Indicator 01 Requested state Current state export=true name=DispPkBrkInd10_Rq_Stat prio=1 dataSetName=std dataClassType=initIO dataClassName=initIO unit='-' description='0,1,2,3 / not requested, requested, res, sna (Display Park(ing) Brake(ing) Indication/Indicator 01 Requested state Current state': pneAux.DispPkBrkInd10_Rq_Stat_0 [-]"; p80 "DispPkBrkInd11_Rq_Stat, 0,1,2,3 / not requested, requested, res, sna (Display Park(ing) Brake(ing) Indication/Indicator 01 Requested state Current state export=true name=DispPkBrkInd11_Rq_Stat prio=1 dataSetName=std dataClassType=initIO dataClassName=initIO unit='-' description='0,1,2,3 / not requested, requested, res, sna (Display Park(ing) Brake(ing) Indication/Indicator 01 Requested state Current state': pneAux.DispPkBrkInd11_Rq_Stat_0 [-]"; p81 "DispPkBrkInd12_Rq_Stat, 0,1,2,3 / not requested, requested, res, sna (Display Park(ing) Brake(ing) Indication/Indicator 01 Requested state Current state export=true name=DispPkBrkInd12_Rq_Stat prio=1 dataSetName=std dataClassType=initIO dataClassName=initIO unit='-' description='0,1,2,3 / not requested, requested, res, sna (Display Park(ing) Brake(ing) Indication/Indicator 01 Requested state Current state': pneAux.DispPkBrkInd12_Rq_Stat_0 [-]"; p82 "DispPkBrkInd13_Rq_Stat, 0,1,2,3 / not requested, requested, res, sna (Display Park(ing) Brake(ing) Indication/Indicator 01 Requested state Current state export=true name=DispPkBrkInd13_Rq_Stat prio=1 dataSetName=std dataClassType=initIO dataClassName=initIO unit='-' description='0,1,2,3 / not requested, requested, res, sna (Display Park(ing) Brake(ing) Indication/Indicator 01 Requested state Current state': pneAux.DispPkBrkInd13_Rq_Stat_0 [-]"; p83 "DispPkBrkInd14_Rq_Stat, 0,1,2,3 / not requested, requested, res, sna (Display Park(ing) Brake(ing) Indication/Indicator 01 Requested state Current state export=true name=DispPkBrkInd14_Rq_Stat prio=1 dataSetName=std dataClassType=initIO dataClassName=initIO unit='-' description='0,1,2,3 / not requested, requested, res, sna (Display Park(ing) Brake(ing) Indication/Indicator 01 Requested state Current state': pneAux.DispPkBrkInd14_Rq_Stat_0 [-]"; p84 "DispPkBrkInd15_Rq_Stat, 0,1,2,3 / not requested, requested, res, sna (Display Park(ing) Brake(ing) Indication/Indicator 01 Requested state Current state export=true name=DispPkBrkInd15_Rq_Stat prio=1 dataSetName=std dataClassType=initIO dataClassName=initIO unit='-' description='0,1,2,3 / not requested, requested, res, sna (Display Park(ing) Brake(ing) Indication/Indicator 01 Requested state Current state': pneAux.DispPkBrkInd15_Rq_Stat_0 [-]"; p85 "DispPkBrkInd16_Rq_Stat, 0,1,2,3 / not requested, requested, res, sna (Display Park(ing) Brake(ing) Indication/Indicator 01 Requested state Current state export=true name=DispPkBrkInd16_Rq_Stat prio=1 dataSetName=std dataClassType=initIO dataClassName=initIO unit='-' description='0,1,2,3 / not requested, requested, res, sna (Display Park(ing) Brake(ing) Indication/Indicator 01 Requested state Current state': pneAux.DispPkBrkInd16_Rq_Stat_0 [-]"; p86 "DispPkBrkInd17_Rq_Stat, 0,1,2,3 / not requested, requested, res, sna (Display Park(ing) Brake(ing) Indication/Indicator 01 Requested state Current state export=true name=DispPkBrkInd17_Rq_Stat prio=1 dataSetName=std dataClassType=initIO dataClassName=initIO unit='-' description='0,1,2,3 / not requested, requested, res, sna (Display Park(ing) Brake(ing) Indication/Indicator 01 Requested state Current state': pneAux.DispPkBrkInd17_Rq_Stat_0 [-]"; p87 "DispPkBrkInd18_Rq_Stat, 0,1,2,3 / not requested, requested, res, sna (Display Park(ing) Brake(ing) Indication/Indicator 01 Requested state Current state export=true name=DispPkBrkInd18_Rq_Stat prio=1 dataSetName=std dataClassType=initIO dataClassName=initIO unit='-' description='0,1,2,3 / not requested, requested, res, sna (Display Park(ing) Brake(ing) Indication/Indicator 01 Requested state Current state': pneAux.DispPkBrkInd18_Rq_Stat_0 [-]"; p88 "drv_DrS_Rq (init) export=true name=drv_DrS_Rq prio=1 dataSetName=std dataClassType=initIO dataClassName=initIO unit='-' description='drv_DrS_Rq': pneAux.drv_DrS_Rq_0 [-]"; p89 "drv_Knl_Rq (init) export=true name=drv_Knl_Rq prio=1 dataSetName=std dataClassType=initIO dataClassName=initIO unit='-' description='drv_Knl_Rq': pneAux.drv_Knl_Rq_0 [-]"; p90 "drv_PB_Sw_Stat_SATP (init) export=true name=drv_PB_Sw_Stat_SATP prio=1 dataSetName=std dataClassType=initIO dataClassName=initIO unit='-' description='Parking brake button: 0,1,2,3 / Not Pressed, Pressed, ERR, SNA)': pneAux.drv_PB_Sw_Stat_SATP_0 [-]"; p91 "drv_PkBrk (init) export=true name=drv_PkBrk prio=1 dataSetName=std dataClassType=initIO dataClassName=initIO unit='-' description='drv_PkBrk': pneAux.drv_PkBrk_0 [-]"; p92 "drv_PkBrkLever_pos (init) export=true name=drv_PkBrkLever_pos prio=1 dataSetName=std dataClassType=initIO dataClassName=initIO unit=% description='drv_PkBrkLever_pos': pneAux.drv_PkBrkLever_pos_0 [-]"; p93 "drv_Trlr_Air_Sup_Sw_Stat (init) export=true name=drv_Trlr_Air_Sup_Sw_Stat prio=1 dataSetName=std dataClassType=initIO dataClassName=initIO unit='-' description='Trailer Air Supply Switch Status for DTNA Varian: 0,1,2,3 /  Neutral, Pulled (Apply PB), Pushed (Release PB), SNA': pneAux.drv_Trlr_Air_Sup_Sw_Stat_0 [-]"; p94 "ElComp_ActDischarge_Stat, ElComp_ActDischarge_Stat  export=true name=ElComp_ActDischarge_Stat prio=1 dataSetName=std dataClassType=initIO dataClassName=initIO unit='-' description='ElComp_ActDischarge_Stat ': pneAux.ElComp_ActDischarge_Stat_0 [-]"; p95 "ElComp_ActlSpd_Cval, Compressor ON [0 - ON, 1 - OFF] export=true name=ElComp_ActlSpd_Cval prio=1 dataSetName=std dataClassType=initIO dataClassName=initIO unit='rpm' description='Compressor ON [0 - ON, 1 - OFF]': pneAux.ElComp_ActlSpd_Cval_0 [-]"; p96 "ElComp_Backup_Rq, ElComp_Backup_Rq  0,1,2,3 / not requested, requested, ERR, SNA --> disturbed communication export=true name=ElComp_Backup_Rq prio=1 dataSetName=std dataClassType=initIO dataClassName=initIO unit='-' description='ElComp_Backup_Rq  0,1,2,3 / not requested, requested, ERR, SNA --> disturbed communication': pneAux.ElComp_Backup_Rq_0 [-]"; p97 "ElComp_CurrentCons_Cval, ElComp_CurrentCons_Cval  0..50, 51..61,62,63 / 0 .. 50,RES,ERR,SNA export=true name=ElComp_CurrentCons_Cval prio=1 dataSetName=std dataClassType=initIO dataClassName=initIO unit='A' description='ElComp_CurrentCons_Cval  0..50, 51..61,62,63 / 0 .. 50,RES,ERR,SNA': pneAux.ElComp_CurrentCons_Cval_0 [-]"; p98 "ElComp_PwrCons_Cval, ElComp_PwrCons_Cval  0..250,251..253,254,255 /  0..12.5, RES,ERR,SNA (E-Compressor power consumption) export=true name=ElComp_PwrCons_Cval prio=1 dataSetName=std dataClassType=initIO dataClassName=initIO unit='kW' description='ElComp_PwrCons_Cval  0..250,251..253,254,255 /  0..12.5, RES,ERR,SNA (E-Compressor power consumption)': pneAux.ElComp_PwrCons_Cval_0 [-]"; p99 "ElComp_SpdMd_Stat, ElComp_SpdMd_Stat  0,1,2,3 / low, med, high SNA (E-compressor speed mode Current state) export=true name=ElComp_SpdMd_Stat prio=1 dataSetName=std dataClassType=initIO dataClassName=initIO unit='-' description='ElComp_SpdMd_Stat  0,1,2,3 / low, med, high SNA (E-compressor speed mode Current state)': pneAux.ElComp_SpdMd_Stat_0 [-]"; p100 "ElComp_Stat, ElComp_Stat  0,1,2,3 /  off, on err, sna (E-Compressor activation state) export=true name=ElComp_Stat prio=1 dataSetName=std dataClassType=initIO dataClassName=initIO unit='-' description='ElComp_Stat  0,1,2,3 /  off, on err, sna (E-Compressor activation state)': pneAux.ElComp_Stat_0 [-]"; p101 "ElComp_Volt_Cval, ElComp_Volt_Cval  0..250,251..253,254,255 /  0..1000, RES,ERR,SNA export=true name=ElComp_Volt_Cval prio=1 dataSetName=std dataClassType=initIO dataClassName=initIO unit='V' description='ElComp_Volt_Cval  0..250,251..253,254,255 /  0..1000, RES,ERR,SNA': pneAux.ElComp_Volt_Cval_0 [-]"; p102 "ElLoadProp_Stat_Trlr2,   export=true name=ElLoadProp_Stat_Trlr2 prio=1 dataSetName=std dataClassType=initIO dataClassName=initIO unit='-' description=' ': pneAux.ElLoadProp_Stat_Trlr2_0 [-]"; p103 "ElLoadProp_Stat_Trlr3,   export=true name=ElLoadProp_Stat_Trlr3 prio=1 dataSetName=std dataClassType=initIO dataClassName=initIO unit='-' description=' ': pneAux.ElLoadProp_Stat_Trlr3_0 [-]"; p104 "ElLoadProp_Stat_Trlr4,   export=true name=ElLoadProp_Stat_Trlr4 prio=1 dataSetName=std dataClassType=initIO dataClassName=initIO unit='-' description=' ': pneAux.ElLoadProp_Stat_Trlr4_0 [-]"; p105 "ElLoadProp_Stat_Trlr5,   export=true name=ElLoadProp_Stat_Trlr5 prio=1 dataSetName=std dataClassType=initIO dataClassName=initIO unit='-' description=' ': pneAux.ElLoadProp_Stat_Trlr5_0 [-]"; p106 "ElLoadProp_Stat_Trlr export=true name=ElLoadProp_Stat_Trlr prio=1 dataSetName=std dataClassType=initIO dataClassName=initIO unit='-' description='ElLoadProp_Stat_Trlr': pneAux.ElLoadProp_Stat_Trlr_0 [-]"; p107 "EngRPM_Cval_CPC3 (init) export=true name=EngRPM_Cval_CPC3 prio=1 dataSetName=std dataClassType=initIO dataClassName=initIO unit='-' description='EngRPM_Cval_CPC3': pneAux.EngRPM_Cval_CPC3_0 [-]"; p108 "amb air Temperature (init) export=true name=env_Temperature prio=1 dataSetName=std dataClassType=initIO dataClassName=initIO unit=degC description='env_Temperature': pneAux.env_Temperature_0 [-]"; p109 "Tolerance Band Level AirSpring +/- [mm] export=true name=epsLevel prio=1 dataSetName=pneAux_dummy dataClassType=main dataClassName=main unit='mm' description='Tolerance Level AirSpring +/- [mm]': pneAux.epsLevel [-]"; p110 "Trailer ABS Config (0 - none, 1- ABS, 2 - EBS (incl. ABS))  export=true name=flagTrailerABS prio=1 dataSetName=veh_dummy dataClassType=veh dataClassName=veh unit='' description='Trailer ABS Config (0 - none, 1- ABS, 2 - EBS (incl. ABS))': pneAux.flagTrailerABS [-]"; p111 "hvs_AirCompressor_nEmot (init) export=true name=hvs_AirCompressor_nEmot prio=1 dataSetName=std dataClassType=initIO dataClassName=initIO unit='rpm' description='Air Compressor E-Motor speed': pneAux.hvs_AirCompressor_nEmot_0 [-]"; p112 "hvs_InverterAirCompressor_hvCurrent (init) export=true name=hvs_InverterAirCompressor_hvCurrent prio=1 dataSetName=std dataClassType=initIO dataClassName=initIO unit='A' description='Air compressor inverter hv current': pneAux.hvs_InverterAirCompressor_hvCurrent_0 [-]"; p113 "hvs_InverterAirCompressor_hvVoltage (init) export=true name=hvs_InverterAirCompressor_hvVoltage prio=1 dataSetName=std dataClassType=initIO dataClassName=initIO unit='V' description='Air compressor inverter hv voltage': pneAux.hvs_InverterAirCompressor_hvVoltage_0 [-]"; p114 "kneelingLevel [mm] export=true name=kneelingLevel prio=1 dataSetName=pneAux_dummy dataClassType=main dataClassName=main unit='mm' description='kneelingLevel' : pneAux.kneelingLevel [-]"; p115 "Compressor Speed High [rpm] export=true name=LP_rpmHigh prio=1 dataSetName=pneAux_dummy dataClassType=main dataClassName=main unit='rpm' description='Compressor Speed High [rpm]': pneAux.LP_rpmHigh [-]"; p116 "Compressor Speed Low [rpm] export=true name=LP_rpmLow prio=1 dataSetName=pneAux_dummy dataClassType=main dataClassName=main unit='rpm' description='Compressor Speed Low [rpm]': pneAux.LP_rpmLow [-]"; p117 "mec_veh_AxleLoad1 (init) export=true name=mec_veh_AxleLoad1 prio=1 dataSetName=std dataClassType=initIO dataClassName=initIO unit=kg description='mec_veh_AxleLoad1': pneAux.mec_veh_AxleLoad1_0 [-]"; p118 "mec_veh_AxleLoad2 (init) export=true name=mec_veh_AxleLoad2 prio=1 dataSetName=std dataClassType=initIO dataClassName=initIO unit=kg description='mec_veh_AxleLoad2': pneAux.mec_veh_AxleLoad2_0 [-]"; p119 "mec_veh_AxleLoad3 (init) export=true name=mec_veh_AxleLoad3 prio=1 dataSetName=std dataClassType=initIO dataClassName=initIO unit=kg description='mec_veh_AxleLoad3': pneAux.mec_veh_AxleLoad3_0 [-]"; p120 "mec_veh_AxleLoad4 (init) export=true name=mec_veh_AxleLoad4 prio=1 dataSetName=std dataClassType=initIO dataClassName=initIO unit=kg description='mec_veh_AxleLoad4': pneAux.mec_veh_AxleLoad4_0 [-]"; p121 "mec_veh_TrailerAxleLoad1 (init) export=true name=mec_veh_TrailerAxleLoad1 prio=1 dataSetName=std dataClassType=initIO dataClassName=initIO unit=kg description='mec_veh_TrailerAxleLoad1': pneAux.mec_veh_TrailerAxleLoad1_0 [-]"; p122 "mec_veh_TrailerAxleLoad2 (init) export=true name=mec_veh_TrailerAxleLoad2 prio=1 dataSetName=std dataClassType=initIO dataClassName=initIO unit=kg description='mec_veh_TrailerAxleLoad2': pneAux.mec_veh_TrailerAxleLoad2_0 [-]"; p123 "mec_veh_TrailerAxleLoad3 (init) export=true name=mec_veh_TrailerAxleLoad3 prio=1 dataSetName=std dataClassType=initIO dataClassName=initIO unit=kg description='mec_veh_TrailerAxleLoad3': pneAux.mec_veh_TrailerAxleLoad3_0 [-]"; p124 "mec_veh_transVel export=true name=mec_veh_transVel prio=1 dataSetName=std dataClassType=initIO dataClassName=initIO unit='-' description='mec_veh_transVel': pneAux.mec_veh_transVel_0 [-]"; p125 "MTBVehicleParameter (0-disabled, 1 enabled) export=true name=MTBVehicleParameter  prio=1 dataSetName=pneAux_dummy dataClassType=main dataClassName=main unit='-' description='MTBVehicleParameter (0-disabled, 1 enabled) ': pneAux.MTBVehicleParameter [-]"; p126 "PB_Sw_Stat_SATP, Parking brake button: 0,1,2,3 / Not Pressed, Pressed, ERR, SNA) export=true name=PB_Sw_Stat_SATP prio=1 dataSetName=std dataClassType=initIO dataClassName=initIO unit='-' description='Parking brake button: 0,1,2,3 / Not Pressed, Pressed, ERR, SNA)': pneAux.PB_Sw_Stat_SATP_0 [-]"; p127 "PB_Trlr_Ctrl_Stat (init) (Parking Brake Trailer Control Current state,0:notAvailable,1:Available,2:error,3:SNA) export=true name=PB_Trlr_Ctrl_Stat prio=1 dataSetName=std dataClassType=initIO dataClassName=initIO unit='-' description='PB_Trlr_Ctrl_Stat (Parking Brake Trailer Control Current state,0:notAvailable,1:Available,2:error,3:SNA)': pneAux.PB_Trlr_Ctrl_Stat_0 [-]"; p128 "PBL_Fct_Stat (init) (Parking Brake Lever Function Current state,0:parkingBrake,1:TrailerBrake,2:error,3:SNA) export=true name=PBL_Fct_Stat prio=1 dataSetName=std dataClassType=initIO dataClassName=initIO unit='-' description='PBL_Fct_Stat (Parking Brake Lever Function Current state,0:parkingBrake,1:TrailerBrake,2:error,3:SNA)': pneAux.PBL_Fct_Stat_0 [-]"; p129 "PBL_LvrPosn_Cval (init) Parking Brake Lever Lever Position Current value export=true name=PBL_LvrPosn_Cval prio=1 dataSetName=std dataClassType=initIO dataClassName=initIO unit=% description='PBL_LvrPosn_Cval Parking Brake Lever Lever Position Current value': pneAux.PBL_LvrPosn_Cval_0 [-]"; p130 "PkB_TrlrAirPress_Stat_ICUC (init) export=true name=PkB_TrlrAirPress_Stat_ICUC prio=1 dataSetName=std dataClassType=initIO dataClassName=initIO unit=kPa description='PkB_TrlrAirPress_Stat_ICUC': pneAux.PkB_TrlrAirPress_Stat_ICUC_0 [-]"; p131 "PkBrk_Engg_Stat (init) (Park(ing) Brake(ing) Engaged Current state,0:notActive,1:active,2:error,3:SNA) export=true name=PkBrk_Engg_Stat prio=1 dataSetName=std dataClassType=initIO dataClassName=initIO unit='-' description='PkBrk_Engg_Stat (Park(ing) Brake(ing) Engaged Current state,0:notActive,1:active,2:error,3:SNA)': pneAux.PkBrk_Engg_Stat_0 [-]"; p132 "PkBrk_Stat_EAPU (init) (Parking Brake Current state,0:Disengaged,1:engaged,2:error,3:SNA) export=true name=PkBrk_Stat_EAPU prio=1 dataSetName=std dataClassType=initIO dataClassName=initIO unit='-' description='PkBrk_Stat_EAPU (Parking Brake Current state,0:Disengaged,1:engaged,2:error,3:SNA)': pneAux.PkBrk_Stat_EAPU_0 [-]"; p133 "PkBrk_Stat_SCH (init) (Parking Brake Current state SAM_CHAS,0:Disengaged,1:engaged,2:error,3:SNA) export=true name=PkBrk_Stat_SCH prio=1 dataSetName=std dataClassType=initIO dataClassName=initIO unit='-' description='PkBrk_Stat_SCH (Parking Brake Current state SAM_CHAS,0:Disengaged,1:engaged,2:error,3:SNA)': pneAux.PkBrk_Stat_SCH_0 [-]"; p134 "PkBrkPress_Cval (init) (Parking Brake Pressure Current value) export=true name=PkBrkPress_Cval prio=1 dataSetName=std dataClassType=initIO dataClassName=initIO unit=kPa description='PkBrkPress_Cval (Parking Brake Pressure Current value)': pneAux.PkBrkPress_Cval_0 [-]"; p135 "pne_brk_Axle1_torque_sns export=true name=pne_brk_Axle1_torque_sns prio=1 dataSetName=std dataClassType=initIO dataClassName=initIO unit='-' description='pne_brk_Axle1_torque_sns': pneAux.pne_brk_Axle1_torque_sns_0 [-]"; p136 "pne_brk_Axle2_torque_sns export=true name=pne_brk_Axle2_torque_sns prio=1 dataSetName=std dataClassType=initIO dataClassName=initIO unit='-' description='pne_brk_Axle2_torque_sns': pneAux.pne_brk_Axle2_torque_sns_0 [-]"; p137 "pne_brk_Axle3_torque_sns export=true name=pne_brk_Axle3_torque_sns prio=1 dataSetName=std dataClassType=initIO dataClassName=initIO unit='-' description='pne_brk_Axle3_torque_sns': pneAux.pne_brk_Axle3_torque_sns_0 [-]"; p138 "pne_brk_Axle4_torque_sns export=true name=pne_brk_Axle4_torque_sns prio=1 dataSetName=std dataClassType=initIO dataClassName=initIO unit='-' description='pne_brk_Axle4_torque_sns': pneAux.pne_brk_Axle4_torque_sns_0 [-]"; p139 "pne_brk_BrkWearAALt export=true name=pne_brk_BrkWearAALt prio=1 dataSetName=std dataClassType=initIO dataClassName=initIO unit='%' description='pne_brk_BrkWearAALt': pneAux.pne_brk_BrkWearAALt_0 [-]"; p140 "pne_brk_BrkWearAARt export=true name=pne_brk_BrkWearAARt prio=1 dataSetName=std dataClassType=initIO dataClassName=initIO unit='%' description='pne_brk_BrkWearAARt': pneAux.pne_brk_BrkWearAARt_0 [-]"; p141 "pne_brk_BrkWearFA1Lt export=true name=pne_brk_BrkWearFA1Lt prio=1 dataSetName=std dataClassType=initIO dataClassName=initIO unit='%' description='pne_brk_BrkWearFA1Lt': pneAux.pne_brk_BrkWearFA1Lt_0 [-]"; p142 "pne_brk_BrkWearFA1Rt export=true name=pne_brk_BrkWearFA1Rt prio=1 dataSetName=std dataClassType=initIO dataClassName=initIO unit='%' description='pne_brk_BrkWearFA1Rt': pneAux.pne_brk_BrkWearFA1Rt_0 [-]"; p143 "pne_brk_BrkWearFA2Lt export=true name=pne_brk_BrkWearFA2Lt prio=1 dataSetName=std dataClassType=initIO dataClassName=initIO unit='%' description='pne_brk_BrkWearFA2Lt': pneAux.pne_brk_BrkWearFA2Lt_0 [-]"; p144 "pne_brk_BrkWearFA2Rt export=true name=pne_brk_BrkWearFA2Rt prio=1 dataSetName=std dataClassType=initIO dataClassName=initIO unit='%' description='pne_brk_BrkWearFA2Rt': pneAux.pne_brk_BrkWearFA2Rt_0 [-]"; p145 "pne_brk_BrkWearRA1Lt export=true name=pne_brk_BrkWearRA1Lt prio=1 dataSetName=std dataClassType=initIO dataClassName=initIO unit='%' description='pne_brk_BrkWearRA1Lt': pneAux.pne_brk_BrkWearRA1Lt_0 [-]"; p146 "pne_brk_BrkWearRA1Rt export=true name=pne_brk_BrkWearRA1Rt prio=1 dataSetName=std dataClassType=initIO dataClassName=initIO unit='%' description='pne_brk_BrkWearRA1Rt': pneAux.pne_brk_BrkWearRA1Rt_0 [-]"; p147 "pne_brk_BrkWearRA2Lt export=true name=pne_brk_BrkWearRA2Lt prio=1 dataSetName=std dataClassType=initIO dataClassName=initIO unit='%' description='pne_brk_BrkWearRA2Lt': pneAux.pne_brk_BrkWearRA2Lt_0 [-]"; p148 "pne_brk_BrkWearRA2Rt export=true name=pne_brk_BrkWearRA2Rt prio=1 dataSetName=std dataClassType=initIO dataClassName=initIO unit='%' description='pne_brk_BrkWearRA2Rt': pneAux.pne_brk_BrkWearRA2Rt_0 [-]"; p149 "Compressor ON (1 - ON, 0 - OFF) (init) export=true name=pne_brk_CompON prio=1 dataSetName=std dataClassType=initIO dataClassName=initIO unit='-' description='Compressor ON (1 - ON, 0 - OFF) (init)': pneAux.pne_brk_CompON_0 [-]"; p150 "Pressure (relative) Spring Brake [bar] (init) export=true name=pne_brk_pRelPkBrk prio=1 dataSetName=std dataClassType=initIO dataClassName=initIO unit=bar description='Pressure (relative) Spring Brake [bar] (init) ': pneAux.pne_brk_pRelPkBrk_0 [-]"; p151 "pne_brk_reg_active (init) export=true name=pne_brk_reg_active prio=1 dataSetName=std dataClassType=initIO dataClassName=initIO unit='-' description='Regeneraaton active': pneAux.pne_brk_reg_active_0 [-]"; p152 "wheel speed trailer axle1 left wheel (init) export=true name=pne_brk_rotVel_t1l prio=1 dataSetName=std dataClassType=initIO dataClassName=initIO unit='-' description='wheel speed trailer axle1 left wheel': pneAux.pne_brk_rotVel_t1l_0 [-]"; p153 "wheel speed trailer axle1 right wheel (init) export=true name=pne_brk_rotVel_t1r prio=1 dataSetName=std dataClassType=initIO dataClassName=initIO unit='-' description='wheel speed trailer axle3 right wheel': pneAux.pne_brk_rotVel_t1r_0 [-]"; p154 "wheel speed trailer axle2 left wheel (init) export=true name=pne_brk_rotVel_t2l prio=1 dataSetName=std dataClassType=initIO dataClassName=initIO unit='-' description='wheel speed trailer axle2 left wheel': pneAux.pne_brk_rotVel_t2l_0 [-]"; p155 "wheel speed trailer axle2 right wheel (init) export=true name=pne_brk_rotVel_t2r prio=1 dataSetName=std dataClassType=initIO dataClassName=initIO unit='-' description='wheel speed trailer axle3 right wheel': pneAux.pne_brk_rotVel_t2r_0 [-]"; p156 "wheel speed trailer axle3 left wheel (init) export=true name=pne_brk_rotVel_t3l prio=1 dataSetName=std dataClassType=initIO dataClassName=initIO unit='-' description='wheel speed trailer axle3 left wheel': pneAux.pne_brk_rotVel_t3l_0 [-]"; p157 "wheel speed trailer axle3 right wheel (init) export=true name=pne_brk_rotVel_t3r prio=1 dataSetName=std dataClassType=initIO dataClassName=initIO unit='-' description='wheel speed trailer axle3 right wheel': pneAux.pne_brk_rotVel_t3r_0 [-]"; p158 "pne_brk_Trailer_RV_Front_pAct (init) export=true name=pne_brk_Trailer_RV_Front_pAct prio=1 dataSetName=std dataClassType=initIO dataClassName=initIO unit='-' description='pne_brk_Trailer_RV_Front_pAct'': pneAux.pne_brk_Trailer_RV_Front_pAct_0 [-]"; p159 "pne_brk_Trailer_RV_Rear_pAct (init) export=true name=pne_brk_Trailer_RV_Rear_pAct prio=1 dataSetName=std dataClassType=initIO dataClassName=initIO unit='-' description='pne_brk_Trailer_RV_Rear_pAct'': pneAux.pne_brk_Trailer_RV_Rear_pAct_0 [-]"; p160 "pne_brk_TrailerAxle1_BrakingForce_at8p5bar (init) export=true name=pne_brk_TrailerAxle1_BrakingForce_at8p5bar prio=1 dataSetName=std dataClassType=initIO dataClassName=initIO unit=N description='pne_brk_TrailerAxle1_BrakingForce_at8p5bar': pneAux.pne_brk_TrailerAxle1_BrakingForce_at8p5bar_0 [-]"; p161 "pne_brk_TrailerAxle1_torque_sns export=true name=pne_brk_TrailerAxle1_torque_sns prio=1 dataSetName=std dataClassType=initIO dataClassName=initIO unit='-' description='pne_brk_TrailerAxle1_torque_sns': pneAux.pne_brk_TrailerAxle1_torque_sns_0 [-]"; p162 "pne_brk_TrailerAxle2_BrakingForce_at8p5bar (init) export=true name=pne_brk_TrailerAxle2_BrakingForce_at8p5bar prio=1 dataSetName=std dataClassType=initIO dataClassName=initIO unit=N description='pne_brk_TrailerAxle2_BrakingForce_at8p5bar': pneAux.pne_brk_TrailerAxle2_BrakingForce_at8p5bar_0 [-]"; p163 "pne_brk_TrailerAxle2_torque_sns export=true name=pne_brk_TrailerAxle2_torque_sns prio=1 dataSetName=std dataClassType=initIO dataClassName=initIO unit='-' description='pne_brk_TrailerAxle2_torque_sns': pneAux.pne_brk_TrailerAxle2_torque_sns_0 [-]"; p164 "pne_brk_TrailerAxle3_BrakingForce_at8p5bar (init) export=true name=pne_brk_TrailerAxle3_BrakingForce_at8p5bar prio=1 dataSetName=std dataClassType=initIO dataClassName=initIO unit=N description='pne_brk_TrailerAxle3_BrakingForce_at8p5bar': pneAux.pne_brk_TrailerAxle3_BrakingForce_at8p5bar_0 [-]"; p165 "pne_brk_TrailerAxle3_torque_sns export=true name=pne_brk_TrailerAxle3_torque_sns prio=1 dataSetName=std dataClassType=initIO dataClassName=initIO unit='-' description='pne_brk_TrailerAxle3_torque_sns': pneAux.pne_brk_TrailerAxle3_torque_sns_0 [-]"; p166 "Relative Pressure Tank1 [bar] (init) export=true name=pne_brk_V1_pRel prio=1 dataSetName=std dataClassType=initIO dataClassName=initIO unit=bar description='Relative Pressure Tank1 [bar] (init) ': pneAux.pne_brk_V1_pRel_0 [-]"; p167 "Relative Pressure Tank2 [bar] (init) export=true name=pne_brk_V2_pRel prio=1 dataSetName=std dataClassType=initIO dataClassName=initIO unit=bar description='Relative Pressure Tank2 [bar] (init) ': pneAux.pne_brk_V2_pRel_0 [-]"; p168 "Relative Pressure Tank4 [bar] (init) export=true name=pne_brk_V4_pRel prio=1 dataSetName=std dataClassType=initIO dataClassName=initIO unit=bar description='Relative Pressure Tank4 [bar] (init) ': pneAux.pne_brk_V4_pRel_0 [-]"; p169 "pne_brk_V7_pRel (init) export=true name=pne_brk_V7_pRel prio=1 dataSetName=std dataClassType=initIO dataClassName=initIO unit='bar' description='Relative Pressure Tank7 [bar]': pneAux.pne_brk_V7_pRel_0 [-]"; p170 "Relative Pressure Tank Trailer [bar] (init) export=true name=pne_brk_VTrailer_pRel prio=1 dataSetName=std dataClassType=initIO dataClassName=initIO unit=bar description='Relative Pressure Tank Trailer [bar] (init) ': pneAux.pne_brk_VTrailer_pRel_0 [-]"; p171 "pne_brk_WetLvl_Cntr (init) export=true name=pne_brk_WetLvl_Cntr prio=1 dataSetName=std dataClassType=initIO dataClassName=initIO unit='Nl' description='Calculated Wettnesslevel of the cartridge / Nl': pneAux.pne_brk_WetLvl_Cntr_0 [-]"; p172 "pne_MTBmodusSwAllowed (init) export=true name=pne_MTBmodusSwAllowed prio=1 dataSetName=std dataClassType=initIO dataClassName=initIO unit='-' description='pne_MTBmodusSwAllowed': pneAux.pne_MTBmodusSwAllowed_0 [-]"; p173 "pne_susp_A1_Le_Posn [mm] (init) export=true name=pne_susp_A1_Le_Posn prio=1 dataSetName=std dataClassType=initIO dataClassName=initIO unit='-' description='pne_susp_A1_Le_Posn [mm]': pneAux.pne_susp_A1_Le_Posn_0 [-]"; p174 "pne_susp_A1_Ri_Posn [mm] (init) export=true name=pne_susp_A1_Ri_Posn prio=1 dataSetName=std dataClassType=initIO dataClassName=initIO unit='-' description='pne_susp_A1_Ri_Posn [mm]': pneAux.pne_susp_A1_Ri_Posn_0 [-]"; p175 "pne_susp_A2_Le_Posn [mm] (init) export=true name=pne_susp_A2_Le_Posn prio=1 dataSetName=std dataClassType=initIO dataClassName=initIO unit='-' description='pne_susp_A2_Le_Posn [mm]': pneAux.pne_susp_A2_Le_Posn_0 [-]"; p176 "pne_susp_A2_Ri_Posn [mm] (init) export=true name=pne_susp_A2_Ri_Posn prio=1 dataSetName=std dataClassType=initIO dataClassName=initIO unit='-' description='pne_susp_A2_Ri_Posn [mm]': pneAux.pne_susp_A2_Ri_Posn_0 [-]"; p177 "pne_susp_A3_Le_Posn [mm] (init) export=true name=pne_susp_A3_Le_Posn prio=1 dataSetName=std dataClassType=initIO dataClassName=initIO unit='-' description='pne_susp_A3_Le_Posn [mm]': pneAux.pne_susp_A3_Le_Posn_0 [-]"; p178 "pne_susp_A3_Ri_Posn [mm] (init) export=true name=pne_susp_A3_Ri_Posn prio=1 dataSetName=std dataClassType=initIO dataClassName=initIO unit='-' description='pne_susp_A3_Ri_Posn [mm]': pneAux.pne_susp_A3_Ri_Posn_0 [-]"; p179 "pneAux_A1_Le_Rq (init) export=true name=pneAux_A1_Le_Rq prio=1 dataSetName=std dataClassType=initIO dataClassName=initIO unit='-' description='pneAux_A1_Le_Rq': pneAux.pneAux_A1_Le_Rq_0 [-]"; p180 "pneAux_A1_LoLi_Rq (init) export=true name=pneAux_A1_LoLi_Rq prio=1 dataSetName=std dataClassType=initIO dataClassName=initIO unit='-' description='pneAux_A1_LoLi_Rq': pneAux.pneAux_A1_LoLi_Rq_0 [-]"; p181 "pneAux_A1_Ri_Rq (init) export=true name=pneAux_A1_Ri_Rq prio=1 dataSetName=std dataClassType=initIO dataClassName=initIO unit='-' description='pneAux_A1_Ri_Rq': pneAux.pneAux_A1_Ri_Rq_0 [-]"; p182 "pneAux_A2_Le_Rq (init) export=true name=pneAux_A2_Le_Rq prio=1 dataSetName=std dataClassType=initIO dataClassName=initIO unit='-' description='pneAux_A2_Le_Rq': pneAux.pneAux_A2_Le_Rq_0 [-]"; p183 "pneAux_A2_LoLi_Rq (init) export=true name=pneAux_A2_LoLi_Rq prio=1 dataSetName=std dataClassType=initIO dataClassName=initIO unit='-' description='pneAux_A2_LoLi_Rq': pneAux.pneAux_A2_LoLi_Rq_0 [-]"; p184 "pneAux_A2_Ri_Rq (init) export=true name=pneAux_A2_Ri_Rq prio=1 dataSetName=std dataClassType=initIO dataClassName=initIO unit='-' description='pneAux_A2_Ri_Rq': pneAux.pneAux_A2_Ri_Rq_0 [-]"; p185 "pneAux_A3_Le_Rq (init) export=true name=pneAux_A3_Le_Rq prio=1 dataSetName=std dataClassType=initIO dataClassName=initIO unit='-' description='pneAux_A3_Le_Rq': pneAux.pneAux_A3_Le_Rq_0 [-]"; p186 "pneAux_A3_LoLi_Rq (init) export=true name=pneAux_A3_LoLi_Rq prio=1 dataSetName=std dataClassType=initIO dataClassName=initIO unit='-' description='pneAux_A3_LoLi_Rq': pneAux.pneAux_A3_LoLi_Rq_0 [-]"; p187 "pneAux_A3_Ri_Rq (init) export=true name=pneAux_A3_Ri_Rq prio=1 dataSetName=std dataClassType=initIO dataClassName=initIO unit='-' description='pneAux_A3_Ri_Rq': pneAux.pneAux_A3_Ri_Rq_0 [-]"; p188 "pneAux_Axle1_load (init) export=true name=pneAux_Axle1_load prio=1 dataSetName=std dataClassType=initIO dataClassName=initIO unit=kg description='pneAux_Axle1_load': pneAux.pneAux_Axle1_load_0 [-]"; p189 "pneAux_Axle2_load (init) export=true name=pneAux_Axle2_load prio=1 dataSetName=std dataClassType=initIO dataClassName=initIO unit=kg description='pneAux_Axle2_load': pneAux.pneAux_Axle2_load_0 [-]"; p190 "pneAux_Axle3_load (init) export=true name=pneAux_Axle3_load prio=1 dataSetName=std dataClassType=initIO dataClassName=initIO unit=kg description='pneAux_Axle3_load': pneAux.pneAux_Axle3_load_0 [-]"; p191 "pneAux_Axle4_load (init) export=true name=pneAux_Axle4_load prio=1 dataSetName=std dataClassType=initIO dataClassName=initIO unit=kg description='pneAux_Axle4_load': pneAux.pneAux_Axle4_load_0 [-]"; p192 "pneAux_Drs_Rq (init) export=true name=pneAux_Drs_Rq prio=1 dataSetName=std dataClassType=initIO dataClassName=initIO unit='-' description='pneAux_Drs_Rq': pneAux.pneAux_Drs_Rq_0 [-]"; p193 "pneAux_EAPU_overrun (init) export=true name=pneAux_EAPU_overrun prio=1 dataSetName=std dataClassType=initIO dataClassName=initIO unit='-' description='pneAux_EAPU_overrun (init)': pneAux.pneAux_EAPU_overrun_0 [-]"; p194 "pneAux_mass_Tractor (init) export=true name=pneAux_mass_Tractor prio=1 dataSetName=std dataClassType=initIO dataClassName=initIO unit=kg description='pneAux_mass_Tractor': pneAux.pneAux_mass_Tractor_0 [-]"; p195 "pneAux_mass_Trailer (init) export=true name=pneAux_mass_Trailer prio=1 dataSetName=std dataClassType=initIO dataClassName=initIO unit=kg description='pneAux_mass_Trailer': pneAux.pneAux_mass_Trailer_0 [-]"; p196 "pneAux_pSoll_TCV_p43 (init) export=true name=pneAux_pSoll_TCV_p43 prio=1 dataSetName=std dataClassType=initIO dataClassName=initIO unit='-' description='pneAux_pSoll_TCV_p43 (init)': pneAux.pneAux_pSoll_TCV_p43_0 [-]"; p197 "pneAux_pSollPkBrk (init) export=true name=pneAux_pSollPkBrk prio=1 dataSetName=std dataClassType=initIO dataClassName=initIO unit='-' description='pneAux_pSollPkBrk (init)': pneAux.pneAux_pSollPkBrk_0 [-]"; p198 "pneAux_SumBrakingForces_Tractor (init) export=true name=pneAux_SumBrakingForces_Tractor prio=1 dataSetName=std dataClassType=initIO dataClassName=initIO unit=N description='pneAux_SumBrakingForces_Tractor': pneAux.pneAux_SumBrakingForces_Tractor_0 [-]"; p199 "pneAux_SumBrakingForces_Trailer (init) export=true name=pneAux_SumBrakingForces_Trailer prio=1 dataSetName=std dataClassType=initIO dataClassName=initIO unit=N description='pneAux_SumBrakingForces_Trailer': pneAux.pneAux_SumBrakingForces_Trailer_0 [-]"; p200 "pneAux_TCV_pDmd_Front_Left (init) export=true name=pneAux_TCV_pDmd_Front_Left prio=1 dataSetName=std dataClassType=initIO dataClassName=initIO unit='-' description='pneAux_TCV_pDmd_Front_Right': pneAux.pneAux_TCV_pDmd_Front_Left_0 [-]"; p201 "pneAux_TCV_pDmd_Front_Right (init) export=true name=pneAux_TCV_pDmd_Front_Right prio=1 dataSetName=std dataClassType=initIO dataClassName=initIO unit='-' description='pneAux_TCV_pDmd_Front_Right': pneAux.pneAux_TCV_pDmd_Front_Right_0 [-]"; p202 "pneAux_TCV_pDmd_Rear_Left (init) export=true name=pneAux_TCV_pDmd_Rear_Left prio=1 dataSetName=std dataClassType=initIO dataClassName=initIO unit='-' description='pneAux_TCV_pDmd_Front_Right': pneAux.pneAux_TCV_pDmd_Rear_Left_0 [-]"; p203 "pneAux_TCV_pDmd_Rear_Right (init) export=true name=pneAux_TCV_pDmd_Rear_Right prio=1 dataSetName=std dataClassType=initIO dataClassName=initIO unit='-' description='pneAux_TCV_pDmd_Front_Right': pneAux.pneAux_TCV_pDmd_Rear_Right_0 [-]"; p204 "pneAux_trailerAxle1_left_stABSInValve export=true name=pneAux_trailerAxle1_left_stABSInValve prio=1 dataSetName=std dataClassType=initIO dataClassName=initIO unit='-' description='pneAux_trailerAxle1_left_stABSInValve': pneAux.pneAux_trailerAxle1_left_stABSInValve_0 [-]"; p205 "pneAux_trailerAxle1_left_stABSOutValve export=true name=pneAux_trailerAxle1_left_stABSOutValve prio=1 dataSetName=std dataClassType=initIO dataClassName=initIO unit='-' description='pneAux_trailerAxle1_left_stABSOutValve': pneAux.pneAux_trailerAxle1_left_stABSOutValve_0 [-]"; p206 "pneAux_trailerAxle1_load (init) export=true name=pneAux_trailerAxle1_load prio=1 dataSetName=std dataClassType=initIO dataClassName=initIO unit=kg description='pneAux_trailerAxle1_load': pneAux.pneAux_trailerAxle1_load_0 [-]"; p207 "pneAux_trailerAxle1_right_stABSInValve export=true name=pneAux_trailerAxle1_right_stABSInValve prio=1 dataSetName=std dataClassType=initIO dataClassName=initIO unit='-' description='pneAux_trailerAxle1_right_stABSInValve': pneAux.pneAux_trailerAxle1_right_stABSInValve_0 [-]"; p208 "pneAux_trailerAxle1_right_stABSOutValve export=true name=pneAux_trailerAxle1_right_stABSOutValve prio=1 dataSetName=std dataClassType=initIO dataClassName=initIO unit='-' description='pneAux_trailerAxle1_right_stABSOutValve': pneAux.pneAux_trailerAxle1_right_stABSOutValve_0 [-]"; p209 "pneAux_trailerAxle2_left_stABSInValve export=true name=pneAux_trailerAxle2_left_stABSInValve prio=1 dataSetName=std dataClassType=initIO dataClassName=initIO unit='-' description='pneAux_trailerAxle2_left_stABSInValve': pneAux.pneAux_trailerAxle2_left_stABSInValve_0 [-]"; p210 "pneAux_trailerAxle2_left_stABSOutValve export=true name=pneAux_trailerAxle2_left_stABSOutValve prio=1 dataSetName=std dataClassType=initIO dataClassName=initIO unit='-' description='pneAux_trailerAxle2_left_stABSOutValve': pneAux.pneAux_trailerAxle2_left_stABSOutValve_0 [-]"; p211 "pneAux_trailerAxle2_load (init) export=true name=pneAux_trailerAxle2_load prio=1 dataSetName=std dataClassType=initIO dataClassName=initIO unit=kg description='pneAux_trailerAxle2_load': pneAux.pneAux_trailerAxle2_load_0 [-]"; p212 "pneAux_trailerAxle2_right_stABSInValve export=true name=pneAux_trailerAxle2_right_stABSInValve prio=1 dataSetName=std dataClassType=initIO dataClassName=initIO unit='-' description='pneAux_trailerAxle2_right_stABSInValve': pneAux.pneAux_trailerAxle2_right_stABSInValve_0 [-]"; p213 "pneAux_trailerAxle2_right_stABSOutValve export=true name=pneAux_trailerAxle2_right_stABSOutValve prio=1 dataSetName=std dataClassType=initIO dataClassName=initIO unit='-' description='pneAux_trailerAxle2_right_stABSOutValve': pneAux.pneAux_trailerAxle2_right_stABSOutValve_0 [-]"; p214 "pneAux_trailerAxle3_left_stABSInValve export=true name=pneAux_trailerAxle3_left_stABSInValve prio=1 dataSetName=std dataClassType=initIO dataClassName=initIO unit='-' description='pneAux_trailerAxle3_left_stABSInValve': pneAux.pneAux_trailerAxle3_left_stABSInValve_0 [-]"; p215 "pneAux_trailerAxle3_left_stABSOutValve export=true name=pneAux_trailerAxle3_left_stABSOutValve prio=1 dataSetName=std dataClassType=initIO dataClassName=initIO unit='-' description='pneAux_trailerAxle3_left_stABSOutValve': pneAux.pneAux_trailerAxle3_left_stABSOutValve_0 [-]"; p216 "pneAux_trailerAxle3_load (init) export=true name=pneAux_trailerAxle3_load prio=1 dataSetName=std dataClassType=initIO dataClassName=initIO unit=kg description='pneAux_trailerAxle3_load': pneAux.pneAux_trailerAxle3_load_0 [-]"; p217 "pneAux_trailerAxle3_right_stABSInValve export=true name=pneAux_trailerAxle3_right_stABSInValve prio=1 dataSetName=std dataClassType=initIO dataClassName=initIO unit='-' description='pneAux_trailerAxle3_right_stABSInValve': pneAux.pneAux_trailerAxle3_right_stABSInValve_0 [-]"; p218 "pneAux_trailerAxle3_right_stABSOutValve export=true name=pneAux_trailerAxle3_right_stABSOutValve prio=1 dataSetName=std dataClassType=initIO dataClassName=initIO unit='-' description='pneAux_trailerAxle3_right_stABSOutValve': pneAux.pneAux_trailerAxle3_right_stABSOutValve_0 [-]"; p219 "Compressor ON (1 - ON, 0 - OFF) (init) export=true name=PressAir_Rq prio=1 dataSetName=std dataClassType=initIO dataClassName=initIO unit='-' description='Compressor ON (1 - ON, 0 - OFF) (init)': pneAux.PressAir_Rq_0 [-]"; p220 "Compressor ON (1 - ON, 0 - OFF) (init) export=true name=PressAir_Rq_ICUC prio=1 dataSetName=std dataClassType=initIO dataClassName=initIO unit='-' description='Compressor ON (1 - ON, 0 - OFF) (init)': pneAux.PressAir_Rq_ICUC_0 [-]"; p221 "PressAir_Rq_SATP, Compressor ON [0 - ON, 1 - OFF] export=true name=PressAir_Rq_SATP prio=1 dataSetName=std dataClassType=initIO dataClassName=initIO unit='-' description='Compressor ON [0 - ON, 1 - OFF]': pneAux.PressAir_Rq_SATP_0 [-]"; p222 "Switching Pressure High to Low Comp. Speed [bar] export=true name=pSwitch_bar prio=1 dataSetName=pneAux_dummy dataClassType=main dataClassName=main unit=bar description='Switching Pressure High to Low Comp. Speed [bar]': pneAux.pSwitch_bar [-]"; p223 "Dyn. Wheel Radius Front Axle [mm] export=true name=rdynFA prio=1 dataSetName=veh_dummy dataClassType=veh dataClassName=veh unit='mm' description='Dyn. Wheel Radius Front Axle [mm]': pneAux.rdynFA [-]"; p224 "Dyn. Wheel Radius Rear Axle [mm] export=true name=rdynRA prio=1 dataSetName=veh_dummy dataClassType=veh dataClassName=veh unit='mm' description='Dyn. Wheel Radius Rear Axle [mm]': pneAux.rdynRA [-]"; p225 "Dyn. Wheel Radius Trailer Axle [mm] export=true name=rdynTA prio=1 dataSetName=veh_dummy dataClassType=veh dataClassName=veh unit='mm' description='Dyn. Wheel Radius Trailer Axle [mm]': pneAux.rdynTA [-]"; p226 "RedWarn_Rq_Trlr2, Red Warning Request Trailer,0:noFailureIndicated,1:FailureIndicated,2:WariningSignalFlashing,3:SNA export=true name=RedWarn_Rq_Trlr2 prio=1 dataSetName=std dataClassType=initIO dataClassName=initIO unit='-' description='Red Warning Request Trailer,0:noFailureIndicated,1:FailureIndicated,2:WariningSignalFlashing,3:SNA': pneAux.RedWarn_Rq_Trlr2_0 [-]"; p227 "RedWarn_Rq_Trlr3,   export=true name=RedWarn_Rq_Trlr3 prio=1 dataSetName=std dataClassType=initIO dataClassName=initIO unit='-' description=' ': pneAux.RedWarn_Rq_Trlr3_0 [-]"; p228 "RedWarn_Rq_Trlr4,   export=true name=RedWarn_Rq_Trlr4 prio=1 dataSetName=std dataClassType=initIO dataClassName=initIO unit='-' description=' ': pneAux.RedWarn_Rq_Trlr4_0 [-]"; p229 "RedWarn_Rq_Trlr5,   export=true name=RedWarn_Rq_Trlr5 prio=1 dataSetName=std dataClassType=initIO dataClassName=initIO unit='-' description=' ': pneAux.RedWarn_Rq_Trlr5_0 [-]"; p230 "RedWarn_Rq_Trlr export=true name=RedWarn_Rq_Trlr prio=1 dataSetName=std dataClassType=initIO dataClassName=initIO unit='-' description='RedWarn_Rq_Trlr': pneAux.RedWarn_Rq_Trlr_0 [-]"; p231 "Step Size ABS [s] export=true name=stepSize prio=1 dataSetName=veh_dummy dataClassType=veh dataClassName=veh unit='s' description='step size [s]': pneAux.stepSize [s]"; p232 "SuspAirPress_Stat_SATP,   export=true name=SuspAirPress_Stat_SATP prio=1 dataSetName=std dataClassType=initIO dataClassName=initIO unit='-' description=' ': pneAux.SuspAirPress_Stat_SATP_0 [-]"; p233 "TBL_LvrPosn_Cval, Lever: 0..100, 101..253,254,255 / 0..100, RES,ERR,SNA export=true name=TBL_LvrPosn_Cval prio=1 dataSetName=std dataClassType=initIO dataClassName=initIO unit='%' description='Lever: 0..100, 101..253,254,255 / 0..100, RES,ERR,SNA': pneAux.TBL_LvrPosn_Cval_0 [-]"; p234 "Minimum Compressor Power-On Time [s] export=true name=tDelay prio=1 dataSetName=pneAux_dummy dataClassType=main dataClassName=main unit='s' description='Minimum Compressor Power-On Time [s]': pneAux.tDelay [-]"; p235 "Velocity Offset L1o (km/h) export=true name=TrailerABS_L1o prio=1 dataSetName=veh_dummy dataClassType=veh dataClassName=veh unit='km/h' description='Velocity Offset L1o (km/h)': pneAux.TrailerABS_L1o [-]"; p236 "Speed Fraction for Threshold Speed 1 (0.01%) export=true name=TrailerABS_L1v prio=1 dataSetName=veh_dummy dataClassType=veh dataClassName=veh unit='' description='Speed Fraction for Threshold Speed 1 (0.01%)': pneAux.TrailerABS_L1v [-]"; p237 "Velocity Offset L2o (km/h) export=true name=TrailerABS_L2o prio=1 dataSetName=veh_dummy dataClassType=veh dataClassName=veh unit='km/h' description='Velocity Offset L2o (km/h)': pneAux.TrailerABS_L2o [-]"; p238 "Speed Fraction for Threshold Speed 2 (0.01%) export=true name=TrailerABS_L2v prio=1 dataSetName=veh_dummy dataClassType=veh dataClassName=veh unit='' description='Speed Fraction for Threshold Speed 2 (0.01%)': pneAux.TrailerABS_L2v [-]"; p239 "Decceleration Threshold in [g] export=true name=TrailerABS_MinusB prio=1 dataSetName=veh_dummy dataClassType=veh dataClassName=veh unit='' description='Decceleration Threshold in [g]': pneAux.TrailerABS_MinusB [-]"; p240 "Acceleration Threshold in [g] export=true name=TrailerABS_PlusB prio=1 dataSetName=veh_dummy dataClassType=veh dataClassName=veh unit='' description='Decceleration Threshold in [g]': pneAux.TrailerABS_PlusB [-]"; p241 "Upper Acceleration Threshold in [g] export=true name=TrailerABS_PlusOB prio=1 dataSetName=veh_dummy dataClassType=veh dataClassName=veh unit='' description='Upper Acceleration Threshold in [g]': pneAux.TrailerABS_PlusOB [-]"; p242 "Holding Time [ms] export=true name=TrailerABS_THe prio=1 dataSetName=veh_dummy dataClassType=veh dataClassName=veh unit='ms' description='Holding Time [ms]': pneAux.TrailerABS_THe [-]"; p243 "Holding Time for Pulsating Pressure Build-Up [ms] export=true name=TrailerABS_TPulHold prio=1 dataSetName=veh_dummy dataClassType=veh dataClassName=veh unit='ms' description='Holding Time for Pulsating Pressure Build-Up [ms]': pneAux.TrailerABS_TPulHold [-]"; p244 "Opening Time for Pulsating Pressure Build-Up [ms] export=true name=TrailerABS_TPulOpen prio=1 dataSetName=veh_dummy dataClassType=veh dataClassName=veh unit='ms' description='Opening Time for Pulsating Pressure Build-Up [ms]': pneAux.TrailerABS_TPulOpen [-]"; p245 "Minimum Velocity for ABS Activity [km/h] export=true name=TrailerABS_vMin_kmh prio=1 dataSetName=veh_dummy dataClassType=veh dataClassName=veh unit='km/h' description='Minimum Velocity for ABS Activity [km/h]': pneAux.TrailerABS_vMin_kmh [-]"; p246 "Trlr_Air_Sup_Sw_Stat, Trailer Air Supply Switch Status for DTNA Varian: 0,1,2,3 /  Neutral, Pulled (Apply PB), Pushed (Release PB), SNA export=true name=Trlr_Air_Sup_Sw_Stat prio=1 dataSetName=std dataClassType=initIO dataClassName=initIO unit='-' description='Trailer Air Supply Switch Status for DTNA Varian: 0,1,2,3 /  Neutral, Pulled (Apply PB), Pushed (Release PB), SNA': pneAux.Trlr_Air_Sup_Sw_Stat_0 [-]"; p247 "Trlr_Air_Supply_Press_Cval, 0..250,251..253,254,255 / 0..2000, RES,ERR,SNA export=true name=Trlr_Air_Supply_Press_Cval prio=1 dataSetName=std dataClassType=initIO dataClassName=initIO unit='kPa' description='0..250,251..253,254,255 / 0..2000, RES,ERR,SNA': pneAux.Trlr_Air_Supply_Press_Cval_0 [-]"; p248 "ABS control active: 0 passive / 1 active / 2 res / 3 SNA (init) export=true name=VehABS_Stat_Trlr prio=1 dataSetName=std dataClassType=initIO dataClassName=initIO unit='-' description='ABS control active: 0 passive / 1 active / 2 res / 3 SNA': pneAux.VehABS_Stat_Trlr_0 [-]"; p249 "Wheel based Vehicel Speed Current Value Trailer (init) export=true name=VehSpd1_Cval_Trlr prio=1 dataSetName=std dataClassType=initIO dataClassName=initIO unit='-' description='Wheel based Vehicel Speed Current Value Trailer': pneAux.VehSpd1_Cval_Trlr_0 [-]"; p250 "WetLvlCntr_Cval_SATP, Cartridge wettness level / Normliter: 0..250, 254, 255 / 0..62500 physicalisch , ERR, SNA   export=true name=WetLvlCntr_Cval_SATP prio=1 dataSetName=std dataClassType=initIO dataClassName=initIO unit='l' description='Cartridge wettness level / Normliter: 0..250, 254, 255 / 0..62500 physicalisch , ERR, SNA  ': pneAux.WetLvlCntr_Cval_SATP_0 [-]"; p251 "Axle Loads Trailer export=true name=axleLoadTrailer_kg prio=1 dataSetName=veh_dummy dataClassType=veh dataClassName=veh unit=kg description='Axle Loads Trailer': pneAux.axleLoadTrailer_kg [-]"; p252 "Axle Loads Vehicle export=true name=axleLoadVehicle_kg prio=1 dataSetName=veh_dummy dataClassType=veh dataClassName=veh unit=kg description='Axle Loads Vehicle': pneAux.axleLoadVehicle_kg [-]"; p253 "Brake Circuit Configuration [A1, A2, A3, A4] (0-Dummy, 1-Front, 2-Rear, 3-Middle(Bus)) export=true name=brkCircuit prio=1 dataSetName=veh_dummy dataClassType=veh dataClassName=veh unit='-' description='Brake Circuit Configuration [A1, A2, A3, A4] (0-Dummy, 1-Front, 2-Rear, 3-Middle(Bus))': pneAux.brkCircuit [-]"; p254 "Brake Circuit Configuration {TA1, TA2, TA3} [0-Dummy, 1-Front, 2-Rear] export=true name=brkCircuitTrailer prio=1 dataSetName=veh_dummy dataClassType=veh dataClassName=veh unit='-' description='Brake Circuit Configuration Trailer {TA1, TA2, TA3} [0-Dummy, 1-Front, 2-Rear]': pneAux.brkCircuitTrailer [-]"; p255 "Trailer Control Active / Trailer can brake {flag, x1, x2, x3, x4, x5, y1, y2, y3, y4, y5} (flag: 0 - no, 1- yes ALB lower limit, 2- yes ALB normal, 3- yes ALB upper limit , 4 - yes without ALB, 5 - with characteristics {{x1 ...x5},{y1...y5}) export=true name=flagTrailerControlActive prio=1 dataSetName=veh_dummy dataClassType=veh dataClassName=veh unit='-' description='Trailer Control Active / Trailer can brake {flag, x1, x2, x3, x4, x5, y1, y2, y3, y4, y5} (flag: 0 - no, 1- yes ALB lower limit, 2- yes ALB normal, 3- yes ALB upper limit , 4 - yes without ALB, 5 - with characteristics {{x1 ...x5},{y1...y5})': pneAux.flagTrailerControlActive [-]"; p256 "application pressure of trailer axles [TA1, TA2, TA3] [bar] export=true name=pAppCyl_Trailer prio=1 dataSetName=veh_dummy dataClassType=veh dataClassName=veh unit='bar' description='application pressure of trailer axles [TA1, TA2, TA3] [bar]': pneAux.pAppCyl_Trailer [-]"; p257 "Trailer Speed Sensor Axle Position [0-false,1-true] {A1,A2,A3} export=true name=speedSensorPosnTrailer prio=1 dataSetName=veh_dummy dataClassType=veh dataClassName=veh unit='' description='Trailer Speed Sensor Axle Position [0-false,1-true] {A1,A2,A3}': pneAux.speedSensorPosnTrailer [-]"
